simulink model "VFlexP"  (R2024a)
settings: Solver=ode23tb  StartTime=0.0  StopTime=3  FixedStep=1e-5
model workspace (MAT data in the model file):
  DCop_DCBUCK.op = opcond.OperatingPoint
  DCop_DCBUCK.op.Model_ = 'untitled4'
  DCop_DCBUCK.op.States_(1) = opcond.StatePoint
  DCop_DCBUCK.op.States_(1).Nx_ = 1
  DCop_DCBUCK.op.States_(1).Block_ = 'untitled4/DCBUCK/Integrator'
  DCop_DCBUCK.op.States_(1).x_ = 0.0993111458289
  DCop_DCBUCK.op.States_(2) = opcond.StatePoint
  DCop_DCBUCK.op.States_(2).Nx_ = 1
  DCop_DCBUCK.op.States_(2).Block_ = 'untitled4/DCBUCK/Integrator1'
  DCop_DCBUCK.op.States_(2).x_ = -1.0059432275
  DCop_DCBUCK.op_report = opcond.OperatingReport
  DCop_DCBUCK.op_report.Outputs_ = opcond.OutputReport
  DCop_DCBUCK.op_report.Outputs_.yspec_ = 0.0993111426985
  DCop_DCBUCK.op_report.Outputs_.Block_ = 'untitled4/out_trim1'
  DCop_DCBUCK.op_report.Outputs_.PortWidth_ = 1
  DCop_DCBUCK.op_report.Outputs_.PortNumber_ = NaN
  DCop_DCBUCK.op_report.Outputs_.y_ = 0.0993111458289
  DCop_DCBUCK.op_report.Outputs_.Known_ = 1
  DCop_DCBUCK.op_report.Outputs_.Min_ = -Inf
  DCop_DCBUCK.op_report.Outputs_.Max_ = Inf
  DCop_DCBUCK.op_report.TerminationString_ = 'Operating point specifications were successfully met.'
  DCop_DCBUCK.op_report.OptimizationOutput_.iterations = 1
  DCop_DCBUCK.op_report.OptimizationOutput_.funcCount = 6
  DCop_DCBUCK.op_report.OptimizationOutput_.constrviolation = 8.64996069397e-05
  DCop_DCBUCK.op_report.OptimizationOutput_.stepsize = 2.19887440386
  DCop_DCBUCK.op_report.OptimizationOutput_.algorithm = 'interior-point'
  DCop_DCBUCK.op_report.OptimizationOutput_.firstorderopt = 0
  DCop_DCBUCK.op_report.OptimizationOutput_.cgiterations = 0
  DCop_DCBUCK.op_report.OptimizationOutput_.message = 'Local minimum found that satisfies the constraints.
    | 
    | Optimization completed because the objective function is non-decreasing in 
    | feasible directions, to within the value of the optimality tolerance,
    | and constraints are satisfied to within the value of the constraint tolerance.
    | 
    | <stopping criteria details>
    | 
    | Optimization completed: The relative first-order optimality measure, 0.000000e+00,
    | is less than options.OptimalityTolerance = 1.000000e-06, and the relative maximum constraint
    | violation, 9.451558e-09, is less than options.ConstraintTolerance = 1.000000e-06.'
  DCop_DCBUCK.op_report.OptimizationOutput_.bestfeasible = []
  DCop_DCBUCK.op_report.Model_ = 'untitled4'
  DCop_DCBUCK.op_report.States_(1) = opcond.StateReport
  DCop_DCBUCK.op_report.States_(1).dx_ = 8.64996069397e-05
  DCop_DCBUCK.op_report.States_(1).Nx_ = 1
  DCop_DCBUCK.op_report.States_(1).Block_ = 'untitled4/DCBUCK/Integrator'
  DCop_DCBUCK.op_report.States_(1).x_ = 0.0993111458289
  DCop_DCBUCK.op_report.States_(1).SteadyState_ = 1
  DCop_DCBUCK.op_report.States_(1).dxMin_ = -Inf
  DCop_DCBUCK.op_report.States_(1).dxMax_ = Inf
  DCop_DCBUCK.op_report.States_(1).Known_ = 0
  DCop_DCBUCK.op_report.States_(1).Min_ = -Inf
  DCop_DCBUCK.op_report.States_(1).Max_ = Inf
  DCop_DCBUCK.op_report.States_(2) = opcond.StateReport
  DCop_DCBUCK.op_report.States_(2).dx_ = -1.77018447944e-06
  DCop_DCBUCK.op_report.States_(2).Nx_ = 1
  DCop_DCBUCK.op_report.States_(2).Block_ = 'untitled4/DCBUCK/Integrator1'
  DCop_DCBUCK.op_report.States_(2).x_ = -1.0059432275
  DCop_DCBUCK.op_report.States_(2).SteadyState_ = 1
  DCop_DCBUCK.op_report.States_(2).dxMin_ = -Inf
  DCop_DCBUCK.op_report.States_(2).dxMax_ = Inf
  DCop_DCBUCK.op_report.States_(2).Known_ = 0
  DCop_DCBUCK.op_report.States_(2).Min_ = -Inf
  DCop_DCBUCK.op_report.States_(2).Max_ = Inf
  Grid_CCVSC_idx = [2; 3; 4; 5; 6; 7; 8; 9; 10; 11; 12]
  Grid_CCVSCs = 1
  Grid_CCVSCs_buses = 1
  Grid_CCVSCs_toM = [0 1 0 0 0 0 0 0 0 0 0 0 ... (781 elements, 71x11)]
  Grid_C_Lines = [0 0]
  Grid_Cbuses = [0.00666666666667 0.00666666666667 0.00666666666667]
  Grid_DC.include = 1
  Grid_DC.Nbuses = 1
  Grid_DC.from = []
  Grid_DC.to = []
  Grid_DC.bus = 4
  Grid_DC.v = 1
  Grid_DC.Lines_toM = []
  Grid_DC.Lines_fromM = []
  Grid_DC.R_Lines = []
  Grid_DC.i_branch = []
  Grid_DC.Rbus = 150
  Grid_DC.DC_PESs_buses = 1
  Grid_DC.DC_PESs_toM = 1
  Grid_DC.DC_PESs_Pg = 0.0025
  Grid_DC.DC_VSMs_toM = [0; 0; 1]
  Grid_DC.DC_VSMs_DC_toM = 1
  Grid_DC.DC_VSMs_buses = 3
  Grid_DC.DC_VSMs_DC_buses = 1
  Grid_DC.DC_VSM_dparams.ratio = 1
  Grid_DC.DC_VSM_dparams.type = 1
  Grid_DC.DC_VSM_dparams.Rf = 0.0003
  Grid_DC.DC_VSM_dparams.Lf = 0.0355
  Grid_DC.DC_VSM_dparams.alpha1 = 0.001
  Grid_DC.DC_VSM_dparams.alpha2 = 0.0015
  Grid_DC.DC_VSM_dparams.alpha3 = 0.002
  Grid_DC.DC_VSM_dparams.Gsw = 0
  Grid_DCop_DCBUCK.op = opcond.OperatingPoint
  Grid_DCop_DCBUCK.op.Model_ = 'untitled'
  Grid_DCop_DCBUCK.op.States_(1) = opcond.StatePoint
  Grid_DCop_DCBUCK.op.States_(1).Nx_ = 1
  Grid_DCop_DCBUCK.op.States_(1).Block_ = 'untitled/DCBUCK/Integrator'
  Grid_DCop_DCBUCK.op.States_(1).x_ = 0.297042066445
  Grid_DCop_DCBUCK.op.States_(2) = opcond.StatePoint
  Grid_DCop_DCBUCK.op.States_(2).Nx_ = 1
  Grid_DCop_DCBUCK.op.States_(2).Block_ = 'untitled/DCBUCK/Integrator1'
  Grid_DCop_DCBUCK.op.States_(2).x_ = -1.00698752155
  Grid_DCop_DCBUCK.op_report = opcond.OperatingReport
  Grid_DCop_DCBUCK.op_report.Outputs_ = opcond.OutputReport
  Grid_DCop_DCBUCK.op_report.Outputs_.yspec_ = 0.297042068743
  Grid_DCop_DCBUCK.op_report.Outputs_.Block_ = 'untitled/out_trim1'
  Grid_DCop_DCBUCK.op_report.Outputs_.PortWidth_ = 1
  Grid_DCop_DCBUCK.op_report.Outputs_.PortNumber_ = NaN
  Grid_DCop_DCBUCK.op_report.Outputs_.y_ = 0.297042066445
  Grid_DCop_DCBUCK.op_report.Outputs_.Known_ = 1
  Grid_DCop_DCBUCK.op_report.Outputs_.Min_ = -Inf
  Grid_DCop_DCBUCK.op_report.Outputs_.Max_ = Inf
  Grid_DCop_DCBUCK.op_report.TerminationString_ = 'Operating point specifications were successfully met.'
  Grid_DCop_DCBUCK.op_report.OptimizationOutput_.iterations = 1
  Grid_DCop_DCBUCK.op_report.OptimizationOutput_.funcCount = 6
  Grid_DCop_DCBUCK.op_report.OptimizationOutput_.constrviolation = 8.27288844959e-05
  Grid_DCop_DCBUCK.op_report.OptimizationOutput_.stepsize = 2.12653445023
  Grid_DCop_DCBUCK.op_report.OptimizationOutput_.algorithm = 'interior-point'
  Grid_DCop_DCBUCK.op_report.OptimizationOutput_.firstorderopt = 0
  Grid_DCop_DCBUCK.op_report.OptimizationOutput_.cgiterations = 0
  Grid_DCop_DCBUCK.op_report.OptimizationOutput_.message = 'Local minimum found that satisfies the constraints.
    | 
    | Optimization completed because the objective function is non-decreasing in 
    | feasible directions, to within the value of the optimality tolerance,
    | and constraints are satisfied to within the value of the constraint tolerance.
    | 
    | <stopping criteria details>
    | 
    | Optimization completed: The relative first-order optimality measure, 0.000000e+00,
    | is less than options.OptimalityTolerance = 1.000000e-06, and the relative maximum constraint
    | violation, 8.342696e-09, is less than options.ConstraintTolerance = 1.000000e-06.'
  Grid_DCop_DCBUCK.op_report.OptimizationOutput_.bestfeasible = []
  Grid_DCop_DCBUCK.op_report.Model_ = 'untitled'
  Grid_DCop_DCBUCK.op_report.States_(1) = opcond.StateReport
  Grid_DCop_DCBUCK.op_report.States_(1).dx_ = 8.27288844959e-05
  Grid_DCop_DCBUCK.op_report.States_(1).Nx_ = 1
  Grid_DCop_DCBUCK.op_report.States_(1).Block_ = 'untitled/DCBUCK/Integrator'
  Grid_DCop_DCBUCK.op_report.States_(1).x_ = 0.297042066445
  Grid_DCop_DCBUCK.op_report.States_(1).SteadyState_ = 1
  Grid_DCop_DCBUCK.op_report.States_(1).dxMin_ = -Inf
  Grid_DCop_DCBUCK.op_report.States_(1).dxMax_ = Inf
  Grid_DCop_DCBUCK.op_report.States_(1).Known_ = 0
  Grid_DCop_DCBUCK.op_report.States_(1).Min_ = -Inf
  Grid_DCop_DCBUCK.op_report.States_(1).Max_ = Inf
  Grid_DCop_DCBUCK.op_report.States_(2) = opcond.StateReport
  Grid_DCop_DCBUCK.op_report.States_(2).dx_ = 1.29998784019e-06
  Grid_DCop_DCBUCK.op_report.States_(2).Nx_ = 1
  Grid_DCop_DCBUCK.op_report.States_(2).Block_ = 'untitled/DCBUCK/Integrator1'
  Grid_DCop_DCBUCK.op_report.States_(2).x_ = -1.00698752155
  Grid_DCop_DCBUCK.op_report.States_(2).SteadyState_ = 1
  Grid_DCop_DCBUCK.op_report.States_(2).dxMin_ = -Inf
  Grid_DCop_DCBUCK.op_report.States_(2).dxMax_ = Inf
  Grid_DCop_DCBUCK.op_report.States_(2).Known_ = 0
  Grid_DCop_DCBUCK.op_report.States_(2).Min_ = -Inf
  Grid_DCop_DCBUCK.op_report.States_(2).Max_ = Inf
  Grid_DCop_DC_PES.op = opcond.OperatingPoint
  Grid_DCop_DC_PES.op.Model_ = 'untitled1'
  Grid_DCop_DC_PES.op.States_(1) = opcond.StatePoint
  Grid_DCop_DC_PES.op.States_(1).Nx_ = 1
  Grid_DCop_DC_PES.op.States_(1).Block_ = 'untitled1/DC_PES/Integrator'
  Grid_DCop_DC_PES.op.States_(1).x_ = 0.166666683417
  Grid_DCop_DC_PES.op.States_(2) = opcond.StatePoint
  Grid_DCop_DC_PES.op.States_(2).Nx_ = 1
  Grid_DCop_DC_PES.op.States_(2).Block_ = 'untitled1/DC_PES/Integrator1'
  Grid_DCop_DC_PES.op.States_(2).x_ = 0.166666683333
  Grid_DCop_DC_PES.op_report = opcond.OperatingReport
  Grid_DCop_DC_PES.op_report.Outputs_ = opcond.OutputReport
  Grid_DCop_DC_PES.op_report.Outputs_.yspec_ = 0.166666666667
  Grid_DCop_DC_PES.op_report.Outputs_.Block_ = 'untitled1/out_trim1'
  Grid_DCop_DC_PES.op_report.Outputs_.PortWidth_ = 1
  Grid_DCop_DC_PES.op_report.Outputs_.PortNumber_ = NaN
  Grid_DCop_DC_PES.op_report.Outputs_.y_ = 0.166666683333
  Grid_DCop_DC_PES.op_report.Outputs_.Known_ = 1
  Grid_DCop_DC_PES.op_report.Outputs_.Min_ = -Inf
  Grid_DCop_DC_PES.op_report.Outputs_.Max_ = Inf
  Grid_DCop_DC_PES.op_report.TerminationString_ = 'Operating point specifications were successfully met.'
  Grid_DCop_DC_PES.op_report.OptimizationOutput_.iterations = 1
  Grid_DCop_DC_PES.op_report.OptimizationOutput_.funcCount = 6
  Grid_DCop_DC_PES.op_report.OptimizationOutput_.constrviolation = 1.66666662138e-08
  Grid_DCop_DC_PES.op_report.OptimizationOutput_.stepsize = 1.17851127835
  Grid_DCop_DC_PES.op_report.OptimizationOutput_.algorithm = 'interior-point'
  Grid_DCop_DC_PES.op_report.OptimizationOutput_.firstorderopt = 0
  Grid_DCop_DC_PES.op_report.OptimizationOutput_.cgiterations = 0
  Grid_DCop_DC_PES.op_report.OptimizationOutput_.message = 'Local minimum found that satisfies the constraints.
    | 
    | Optimization completed because the objective function is non-decreasing in 
    | feasible directions, to within the value of the optimality tolerance,
    | and constraints are satisfied to within the value of the constraint tolerance.
    | 
    | <stopping criteria details>
    | 
    | Optimization completed: The relative first-order optimality measure, 0.000000e+00,
    | is less than options.OptimalityTolerance = 1.000000e-06, and the relative maximum constraint
    | violation, 1.666667e-08, is less than options.ConstraintTolerance = 1.000000e-06.'
  Grid_DCop_DC_PES.op_report.OptimizationOutput_.bestfeasible.x = [0.166666683333; 0.166666683417]
  Grid_DCop_DC_PES.op_report.OptimizationOutput_.bestfeasible.fval = 0
  Grid_DCop_DC_PES.op_report.OptimizationOutput_.bestfeasible.constrviolation = 1.66666662138e-08
  Grid_DCop_DC_PES.op_report.OptimizationOutput_.bestfeasible.firstorderopt = 0
  Grid_DCop_DC_PES.op_report.Model_ = 'untitled1'
  Grid_DCop_DC_PES.op_report.States_(1) = opcond.StateReport
  Grid_DCop_DC_PES.op_report.States_(1).Nx_ = 1
  Grid_DCop_DC_PES.op_report.States_(1).Block_ = 'untitled1/DC_PES/Integrator'
  Grid_DCop_DC_PES.op_report.States_(1).x_ = 0.166666683417
  Grid_DCop_DC_PES.op_report.States_(1).SteadyState_ = 1
  Grid_DCop_DC_PES.op_report.States_(1).dxMin_ = -Inf
  Grid_DCop_DC_PES.op_report.States_(1).dxMax_ = Inf
  Grid_DCop_DC_PES.op_report.States_(1).Known_ = 0
  Grid_DCop_DC_PES.op_report.States_(1).Min_ = -Inf
  Grid_DCop_DC_PES.op_report.States_(1).Max_ = Inf
  Grid_DCop_DC_PES.op_report.States_(2) = opcond.StateReport
  Grid_DCop_DC_PES.op_report.States_(2).dx_ = 8.33333402284e-10
  Grid_DCop_DC_PES.op_report.States_(2).Nx_ = 1
  Grid_DCop_DC_PES.op_report.States_(2).Block_ = 'untitled1/DC_PES/Integrator1'
  Grid_DCop_DC_PES.op_report.States_(2).x_ = 0.166666683333
  Grid_DCop_DC_PES.op_report.States_(2).SteadyState_ = 1
  Grid_DCop_DC_PES.op_report.States_(2).dxMin_ = -Inf
  Grid_DCop_DC_PES.op_report.States_(2).dxMax_ = Inf
  Grid_DCop_DC_PES.op_report.States_(2).Known_ = 0
  Grid_DCop_DC_PES.op_report.States_(2).Min_ = -Inf
  Grid_DCop_DC_PES.op_report.States_(2).Max_ = Inf
  Grid_DFIGs = 1
  Grid_DFIGs_buses = 1
  Grid_DGs = "GFr"
  Grid_From_buses = [1 2]
  Grid_GFls = 1
  Grid_GFls_buses = 1
  Grid_GFr_idx = 1
  Grid_GFrs = 1
  Grid_GFrs_buses = 1
  Grid_GFrs_toM = [1; 0; 0]
  Grid_IG_idx = 2
  Grid_IGs = 1
  Grid_IGs_buses = 1
  Grid_IGs_toM = [0; 1]
  Grid_L_Lines = [0.05 0.05]
  Grid_L_Loads = 0
  Grid_Lines_fromM : object (value not decoded)
  Grid_Lines_toM : object (value not decoded)
  Grid_Load_buses = []
  Grid_Load_busesDC = []
  Grid_MSGs = 1
  Grid_MSGs_buses = 1
  Grid_Nbuses = 3
  Grid_PQ_gen = 3
  Grid_Ploads = []
  Grid_PloadsDC = []
  Grid_Ps_lf = -0.138475313333
  Grid_Qloads = []
  Grid_Qs_lf = 0.00594619333333
  Grid_R_Lines = [0.005 0.005]
  Grid_R_Loads = 0
  Grid_R_Loads_DC = 0
  Grid_Rcf = [150 150 150]
  Grid_SCs = 1
  Grid_SCs_buses = 1
  Grid_SG_idx = 1
  Grid_SGs = 1
  Grid_SGs_buses = 1
  Grid_SGs_toM = [1; 0]
  Grid_To_buses = [2 3]
  Grid_VCVSC_idx = [1; 2; 3; 4; 5; 6; 7; 8; 9; 10; 11; 12]
  Grid_VCVSCs = 1
  Grid_VCVSCs_buses = [1; 2; 3; 6; 8; 9; 12; 58; 59; 60; 63; 65]
  Grid_VCVSCs_toM = [1 0 0 0 0 0 0 0 0 0 0 0 ... (852 elements, 71x12)]
  Grid_VSM_idx = 2
  Grid_VSMs = 1
  Grid_VSMs_buses = 1
  Grid_VSMs_toM = [0; 1]
  Grid_admitt_matrix = [1.9801990198-19.801979198i  -1.9801980198+19.801980198i; -1.9801980198+19.801980198i  1.9801990198-19.801979198i]
  Grid_admitt_matrix_noloads = [1.9801990198-19.801979198i  -1.9801980198+19.801980198i; -1.9801980198+19.801980198i  1.9801990198-19.801979198i]
  Grid_bus = [1; 2; 3]
  Grid_busDC_complexity = 1
  Grid_busDC_complexity_PF = 2
  Grid_bus_complexity = [1 1 1]
  Grid_bus_complexity_PF = [1 1 1]
  Grid_buses_lf = 1
  Grid_conductance_matrix = 0.00666666666667
  Grid_conductance_matrix_noloads = 0.00666666666667
  Grid_fref.areas = 1
  Grid_fref.ref_units = 1
  Grid_fref.Fb_units = 1
  Grid_fref.buses = [1 1 1]
  Grid_fref.lines = [1 1]
  Grid_fref.loads = []
  Grid_fref.GFr = 1
  Grid_fref.DC_VSM = 1
  Grid_gen_static_params.mBase = 100
  Grid_iPs_lf = -7.22150378958
  Grid_iQs_lf = 168.17482109
  Grid_iadmitt_matrix = [250000.001075-249999.987531i  249999.998575-250000.012531i; 249999.998575-250000.012531i  250000.001075-249999.987531i]
  Grid_iadmitt_matrix_noloads = [250000.001075-249999.987531i  249999.998575-250000.012531i; 249999.998575-250000.012531i  250000.001075-249999.987531i]
  Grid_iconductance_matrix = 150
  Grid_iconductance_matrix_noloads = 150
  Grid_init_OK_bool = 1
  Grid_intconv_PF.include = 1
  Grid_intconv_PF.vmod = 1
  Grid_intconv_PF.vangle = 0.859745829367
  Grid_intconv_PF.P = -0.158700091527
  Grid_intconv_PF.Q = 0.0237163123873
  Grid_intconv_PF.from = [1 2 4]
  Grid_intconv_PF.to = [2 3 3]
  Grid_lf_op.op_report.Outputs(1).y = -0.138475313333
  Grid_lf_op.op_report.Outputs(2).y = 0.00594619333333
  Grid_lf_op.op_report.Outputs(3).y = [-0.145141982765 -0.151760481969]
  Grid_lf_op.op_report.Outputs(4).y = [-0.0126128600915 -0.0193289630611]
  Grid_lf_op.op_report.Outputs(5).y = [1 1.00009506691 0.999887421166]
  Grid_lf_op.op_report.Outputs(6).y = [0 0.00732016343869 0.0150048323525]
  Grid_lineDC_complexity = []
  Grid_lineDC_complexity_PF = []
  Grid_line_complexity = [1 1]
  Grid_line_complexity_PF = [3 3]
  Grid_loadDC_complexity = []
  Grid_loadDC_complexity_PF = []
  Grid_load_complexity = []
  Grid_load_complexity_PF = []
  Grid_opDC_CCVSC.P = [-0.000250314011939 0.0893885558248 -0.0965482172065 -0.839732591503 -0.318845576293 0.332848927017 0.493081958469 0.184553200933]
  Grid_opDC_CCVSC.Q = [-0.0188263035971 0.0721906871944 0.00896391516299 0.324071624692 -0.392719357789 -0.481473754372 -0.41568236758 -0.296587741983]
  Grid_opDC_CCVSC.id_out = [-0.000238257445549 0.0859724063763 -0.0913415354387 -0.807435184137 -0.305115384013 0.332898648568 0.502342982161 0.183243588375]
  Grid_opDC_CCVSC.iq_out = [0.0179195202435 -0.0694317861922 -0.00848050640623 -0.311607331434 0.375807997884 0.481545677758 0.423489678695 0.294483118332]
  Grid_opDC_CCVSC.PId = [-1.21511297231e-05 0.00657688908779 -0.00698762746106 -0.041179194391 -0.023341326877 0.0254667466155 0.0384292381353 0.0140181345107]
  Grid_opDC_CCVSC.PIq = [0.00091389553242 -0.00531153164371 -0.000648758740077 -0.0158919739032 0.0287493118381 0.0368382443485 0.0323969604201 0.0225279585524]
  Grid_opDC_CCVSC.frame = [-0.213709310357 -0.211881545906 -0.207881074849 0 -0.0555827722547 -0.0954948489365 -0.0996472270949 -0.073605567843]
  Grid_opDC_VSM.P = 0.158700091527
  Grid_opDC_VSM.Q = -0.0237163123873
  Grid_opDC_VSM.id_out = 0.158326365965
  Grid_opDC_VSM.iq_out = 0.0260949107001
  Grid_opDC_VSM.frame = 0.0206507879117
  Grid_opDC_VSM.id_in = 0.000111842024523
  Grid_opDC_VSM.iq_in = 1.84334910023e-05
  Grid_opDC_VSM.IP = 0
  Grid_opDC_VSM.iv = -0.000778396280495
  Grid_opGFr.Pd = -0.138475313333
  Grid_opGFr.Qd = 0.00594619333333
  Grid_opGFr.id_out = -0.138475313333
  Grid_opGFr.iq_out = -0.00594619333333
  Grid_opGFr.frame = -0.00139080832243
  Grid_opGFr.vd_c = 0.999921953718
  Grid_opGFr.vq_c = 0
  Grid_opGFr.iV = -7.80462817455e-05
  Grid_opGFr.v = 0.999921953718
  Grid_opGFr.IntConnect = 5
  Grid_opGFr.id_l = -0.138465909469
  Grid_opGFr.iq_l = 0.0938534152333
  Grid_opGFr.PIid = -0.00138465909469
  Grid_opGFr.PIiq = 0.000938534152333
  Grid_opGFr.PIvd = 9.99921953709e-06
  Grid_opGFr.PIvq = 0
  Grid_opVCVSC.Pd = 0
  Grid_opVCVSC.Qd = 0
  Grid_opVCVSC.id_out = [4.77012824674 0.000252372172029 0.387206076232 -0.00669815177796 4.43044477222 -0.00888398142826 2.79473009232 2.18798980312 0.322264460806 -0.0632019138679 -0.0604985051331 -0.0462539180443]
  Grid_opVCVSC.iq_out = [-1.25997186372 0.0149684790164 -0.231751502643 -0.0494644982143 -0.911066731256 -0.0589472249505 -1.80353640382 0.162268294537 -1.0981777606 -0.338765693762 -0.298705341855 -0.251695536875]
  Grid_opVCVSC.frame = [0.0438933282651 -0.0168438196467 -0.0841666076082 -0.134645533542 -0.017373173296 -0.149645793269 -0.137562101317 0.0572176344752 -0.0529798109092 -0.184784853699 -0.200116593784 -0.181975782571]
  Grid_opVCVSC.vd_c = [1.0583892424 1.00985029405 0.987381572831 0.980499160746 1.0168380704 0.980596131031 1.0316409122 1.06159711208 1.05617213999 1.01344616766 1.07304774652 1.09255913271]
  Grid_opVCVSC.vq_c = [6.93889390391e-18 3.46944695195e-18 0 2.77555756156e-17 0 -2.77555756156e-17 0 -6.93889390391e-18 6.93889390391e-18 -2.77555756156e-17 0 2.77555756156e-17]
  Grid_opVCVSC.iV = [0.0183892424009 -0.000149705952964 0.00238157283064 0.00049916074618 0.0118380704031 0.000596131030837 0.0166409121976 0.00159711208293 0.0111721399885 0.00344616765999 0.00304774652066 0.00255913270857]
  Grid_opVCVSC.v = [1.0583892424 1.00985029405 0.987381572831 0.980499160746 1.0168380704 0.980596131031 1.0316409122 1.06159711208 1.05617213999 1.01344616766 1.07304774652 1.09255913271]
  Grid_opVCVSC.id_l = [4.71024831855 1.231783245e-06 0.405319101793 3.52165566611e-06 4.44560451561 4.60461660484e-06 3.01564651745 2.19368980083 0.379967383234 0.000118194487427 8.76348532929e-05 6.10344572474e-05]
  Grid_opVCVSC.iq_l = [-1.36222896789 0.115955635796 -0.0996416062474 0.0481339685791 -0.732278422455 0.0384466913306 -1.30009716484 0.143039154495 -0.973954167095 -0.243266270257 -0.197465537031 -0.146654353471]
  Grid_opVCVSC.PIid = [0.000135655151574 3.5475357456e-11 1.16731901316e-05 1.01423683184e-10 0.00012803341005 1.32612958219e-10 8.68506197027e-05 6.31782662639e-05 1.09430606371e-05 3.40400123789e-09 2.52388377483e-09 1.75779236873e-09]
  Grid_opVCVSC.PIiq = [-3.92321942752e-05 3.33952231093e-06 -2.86967825993e-06 1.38625829508e-06 -2.10896185667e-05 1.10726471032e-06 -3.74427983473e-05 4.11952764945e-06 -2.80498800123e-05 -7.00606858342e-06 -5.68700746649e-06 -4.22364537998e-06]
  Grid_opVCVSC.PIvd = [3.67496264593e-05 3.50642463211e-05 3.42840823902e-05 3.40451097481e-05 3.53068774525e-05 3.40484767719e-05 3.58208650088e-05 3.68610108331e-05 3.66726437489e-05 3.51891030437e-05 3.72586023097e-05 3.79360809968e-05]
  Grid_opVCVSC.PIvq = [-3.85494105773e-15 0 0 0 4.81867632216e-16 0 -2.40933816108e-15 4.81867632216e-16 0 0 -4.81867632216e-16 -4.81867632216e-16]
  Grid_op_CCVSC.op = opcond.OperatingPoint
  Grid_op_CCVSC.op.Model_ = 'untitled'
  Grid_op_CCVSC.op.States_(1) = opcond.StatePoint
  Grid_op_CCVSC.op.States_(1).Nx_ = 11
  Grid_op_CCVSC.op.States_(1).Block_ = 'untitled/CCVSC/LPF/I'
  Grid_op_CCVSC.op.States_(1).x_ = [1.009861943; 0.981291076401; 0.971352962827; 1.00322239915; 0.969168759309; 1.00101830201; 1.05929040967; 1.04339572399; 0.992934596599; 1.04879026715; 1.07220457445]
  Grid_op_CCVSC.op.States_(2) = opcond.StatePoint
  Grid_op_CCVSC.op.States_(2).Nx_ = 11
  Grid_op_CCVSC.op.States_(2).Block_ = 'untitled/CCVSC/LPF1/I'
  Grid_op_CCVSC.op.States_(2).x_ = [-0.0166989844806; -0.085398033397; -0.129897735513; -0.0597487458922; -0.14529940151; -0.167892796173; 0.038779556309; -0.0578823653869; -0.184880740706; -0.211988173785; -0.196156450928]
  Grid_op_CCVSC.op.States_(3) = opcond.StatePoint
  Grid_op_CCVSC.op.States_(3).Nx_ = 11
  Grid_op_CCVSC.op.States_(3).Block_ = 'untitled/CCVSC/LPF2/I'
  Grid_op_CCVSC.op.States_(3).x_ = [1.009861943; 0.981291076401; 0.971352962827; 1.00322239915; 0.969168759309; 1.00101830201; 1.05929040967; 1.04339572399; 0.992934596599; 1.04879026715; 1.07220457445]
  Grid_op_CCVSC.op.States_(4) = opcond.StatePoint
  Grid_op_CCVSC.op.States_(4).Nx_ = 11
  Grid_op_CCVSC.op.States_(4).Block_ = 'untitled/CCVSC/LPF3/I'
  Grid_op_CCVSC.op.States_(4).x_ = [-0.0166989844806; -0.085398033397; -0.129897735513; -0.0597487458926; -0.14529940151; -0.167892796174; 0.0387795563087; -0.0578823653869; -0.184880740706; -0.211988173785; -0.196156450928]
  Grid_op_CCVSC.op.States_(5) = opcond.StatePoint
  Grid_op_CCVSC.op.States_(5).Nx_ = 11
  Grid_op_CCVSC.op.States_(5).Block_ = 'untitled/CCVSC/P'
  Grid_op_CCVSC.op.States_(5).x_ = [1.01727038409e-18; 0.400000000001; -1.80456749167e-13; 4.5000000022; 3.15175961175e-13; 3.10000001288; 2.32400000036; 0.400000000095; -1.95503794004e-12; -3.47571023681e-11; 9.07830100881e-12]
  Grid_op_CCVSC.op.States_(6) = opcond.StatePoint
  Grid_op_CCVSC.op.States_(6).Nx_ = 11
  Grid_op_CCVSC.op.States_(6).Block_ = 'untitled/CCVSC/PLL/dynamic/PLL/I'
  Grid_op_CCVSC.op.States_(6).x_ = [1; 1; 1; 0.999999999991; 1; 0.999999999962; 1; 1; 1; 1; 1]
  Grid_op_CCVSC.op.States_(7) = opcond.StatePoint
  Grid_op_CCVSC.op.States_(7).Nx_ = 11
  Grid_op_CCVSC.op.States_(7).Block_ = 'untitled/CCVSC/PLL/dynamic/frame'
  Grid_op_CCVSC.op.States_(7).x_ = [-0.0165344013704; -0.0868074935304; -0.132939939029; -0.0594865631615; -0.148813342999; -0.166175316605; 0.0365926525094; -0.0554181853462; -0.184088222665; -0.199439311658; -0.180945834503]
  Grid_op_CCVSC.op.States_(8) = opcond.StatePoint
  Grid_op_CCVSC.op.States_(8).Nx_ = 11
  Grid_op_CCVSC.op.States_(8).Block_ = 'untitled/CCVSC/Q'
  Grid_op_CCVSC.op.States_(8).x_ = [-0.015862822257; 0.120252486258; 0.0522438711347; 0.647307088531; 0.0546742450618; 1.36800880468; -0.0931237077542; 1.06159295924; 0.342624354062; 0.31755952052; 0.276277445204]
  Grid_op_CCVSC.op_report = opcond.OperatingReport
  Grid_op_CCVSC.op_report.Outputs_(1) = opcond.OutputReport
  Grid_op_CCVSC.op_report.Outputs_(1).yspec_ = [0.000259673583656; 0.393977793367; -0.0070661813362; 4.43140001829; -0.00827169417353; 2.7891744299; 2.18777108046; 0.325918162006; -0.0620965046483; -0.05879890244; -0.0456136713835]
  Grid_op_CCVSC.op_report.Outputs_(1).Block_ = 'untitled/out_trim1'
  Grid_op_CCVSC.op_report.Outputs_(1).PortWidth_ = 11
  Grid_op_CCVSC.op_report.Outputs_(1).PortNumber_ = NaN
  Grid_op_CCVSC.op_report.Outputs_(1).y_ = [0.000259673583656; 0.393977793229; -0.00706618133531; 4.43139980848; -0.00827169417363; 2.78917339713; 2.18777105686; 0.325918157997; -0.0620965045362; -0.0587989014357; -0.0456136713993]
  Grid_op_CCVSC.op_report.Outputs_(1).Known_ = [1; 1; 1; 1; 1; 1; 1; 1; 1; 1; 1]
  Grid_op_CCVSC.op_report.Outputs_(1).Min_ = [-Inf; -Inf; -Inf; -Inf; -Inf; -Inf; -Inf; -Inf; -Inf; -Inf; -Inf]
  Grid_op_CCVSC.op_report.Outputs_(1).Max_ = [Inf; Inf; Inf; Inf; Inf; Inf; Inf; Inf; Inf; Inf; Inf]
  Grid_op_CCVSC.op_report.Outputs_(2) = opcond.OutputReport
  Grid_op_CCVSC.op_report.Outputs_(2).yspec_ = [0.0157036177884; -0.156831564843; -0.0528396907676; -0.909148054024; -0.0551734384103; -1.8344231967; 0.16800352209; -1.03552070385; -0.3335002201; -0.290901679261; -0.24932744737]
  Grid_op_CCVSC.op_report.Outputs_(2).Block_ = 'untitled/out_trim2'
  Grid_op_CCVSC.op_report.Outputs_(2).PortWidth_ = 11
  Grid_op_CCVSC.op_report.Outputs_(2).PortNumber_ = NaN
  Grid_op_CCVSC.op_report.Outputs_(2).y_ = [0.0157036177884; -0.156831564765; -0.0528396907661; -0.909148031788; -0.0551734384082; -1.83442292878; 0.168003502174; -1.03552070255; -0.333500219896; -0.29090167819; -0.249327447093]
  Grid_op_CCVSC.op_report.Outputs_(2).Known_ = [1; 1; 1; 1; 1; 1; 1; 1; 1; 1; 1]
  Grid_op_CCVSC.op_report.Outputs_(2).Min_ = [-Inf; -Inf; -Inf; -Inf; -Inf; -Inf; -Inf; -Inf; -Inf; -Inf; -Inf]
  Grid_op_CCVSC.op_report.Outputs_(2).Max_ = [Inf; Inf; Inf; Inf; Inf; Inf; Inf; Inf; Inf; Inf; Inf]
  Grid_op_CCVSC.op_report.TerminationString_ = 'Operating point specifications were successfully met.'
  Grid_op_CCVSC.op_report.OptimizationOutput_.iterations = 3
  Grid_op_CCVSC.op_report.OptimizationOutput_.funcCount = 356
  Grid_op_CCVSC.op_report.OptimizationOutput_.constrviolation = 2.89733602665e-05
  Grid_op_CCVSC.op_report.OptimizationOutput_.stepsize = 8.75730946062e-07
  Grid_op_CCVSC.op_report.OptimizationOutput_.algorithm = 'interior-point'
  Grid_op_CCVSC.op_report.OptimizationOutput_.firstorderopt = 0
  Grid_op_CCVSC.op_report.OptimizationOutput_.cgiterations = 0
  Grid_op_CCVSC.op_report.OptimizationOutput_.message = 'Local minimum found that satisfies the constraints.
    | 
    | Optimization completed because the objective function is non-decreasing in 
    | feasible directions, to within the value of the optimality tolerance,
    | and constraints are satisfied to within the value of the constraint tolerance.
    | 
    | <stopping criteria details>
    | 
    | Optimization completed: The relative first-order optimality measure, 0.000000e+00,
    | is less than options.OptimalityTolerance = 1.000000e-06, and the relative maximum constraint
    | violation, 6.438525e-07, is less than options.ConstraintTolerance = 1.000000e-06.'
  Grid_op_CCVSC.op_report.OptimizationOutput_.bestfeasible = []
  Grid_op_CCVSC.op_report.Model_ = 'untitled'
  Grid_op_CCVSC.op_report.States_(1) = opcond.StateReport
  Grid_op_CCVSC.op_report.States_(1).dx_ = [0; -8.881784197e-14; 3.33066907388e-14; 2.35367281221e-12; 6.66133814775e-14; -9.1748830755e-11; 8.881784197e-13; -6.12843109593e-12; 2.33146835171e-13; 1.04360964315e-12; -2.22044604925e-14]
  Grid_op_CCVSC.op_report.States_(1).Nx_ = 11
  Grid_op_CCVSC.op_report.States_(1).Block_ = 'untitled/CCVSC/LPF/I'
  Grid_op_CCVSC.op_report.States_(1).x_ = [1.009861943; 0.981291076401; 0.971352962827; 1.00322239915; 0.969168759309; 1.00101830201; 1.05929040967; 1.04339572399; 0.992934596599; 1.04879026715; 1.07220457445]
  Grid_op_CCVSC.op_report.States_(1).SteadyState_ = [1; 1; 1; 1; 1; 1; 1; 1; 1; 1; 1]
  Grid_op_CCVSC.op_report.States_(1).dxMin_ = [-Inf; -Inf; -Inf; -Inf; -Inf; -Inf; -Inf; -Inf; -Inf; -Inf; -Inf]
  Grid_op_CCVSC.op_report.States_(1).dxMax_ = [Inf; Inf; Inf; Inf; Inf; Inf; Inf; Inf; Inf; Inf; Inf]
  Grid_op_CCVSC.op_report.States_(1).Known_ = [0; 0; 0; 0; 0; 0; 0; 0; 0; 0; 0]
  Grid_op_CCVSC.op_report.States_(1).Min_ = [-Inf; -Inf; -Inf; -Inf; -Inf; -Inf; -Inf; -Inf; -Inf; -Inf; -Inf]
  Grid_op_CCVSC.op_report.States_(1).Max_ = [Inf; Inf; Inf; Inf; Inf; Inf; Inf; Inf; Inf; Inf; Inf]
  Grid_op_CCVSC.op_report.States_(2) = opcond.StateReport
  Grid_op_CCVSC.op_report.States_(2).dx_ = [0; 3.85802501057e-13; 3.80251385934e-13; -3.1668417888e-11; 4.27435864481e-13; -1.02551300785e-10; -2.89226975703e-11; 5.26662047307e-13; -9.99200722163e-14; -2.40363284831e-12; -1.34614541736e-12]
  Grid_op_CCVSC.op_report.States_(2).Nx_ = 11
  Grid_op_CCVSC.op_report.States_(2).Block_ = 'untitled/CCVSC/LPF1/I'
  Grid_op_CCVSC.op_report.States_(2).x_ = [-0.0166989844806; -0.085398033397; -0.129897735513; -0.0597487458922; -0.14529940151; -0.167892796173; 0.038779556309; -0.0578823653869; -0.184880740706; -0.211988173785; -0.196156450928]
  Grid_op_CCVSC.op_report.States_(2).SteadyState_ = [1; 1; 1; 1; 1; 1; 1; 1; 1; 1; 1]
  Grid_op_CCVSC.op_report.States_(2).dxMin_ = [-Inf; -Inf; -Inf; -Inf; -Inf; -Inf; -Inf; -Inf; -Inf; -Inf; -Inf]
  Grid_op_CCVSC.op_report.States_(2).dxMax_ = [Inf; Inf; Inf; Inf; Inf; Inf; Inf; Inf; Inf; Inf; Inf]
  Grid_op_CCVSC.op_report.States_(2).Known_ = [0; 0; 0; 0; 0; 0; 0; 0; 0; 0; 0]
  Grid_op_CCVSC.op_report.States_(2).Min_ = [-Inf; -Inf; -Inf; -Inf; -Inf; -Inf; -Inf; -Inf; -Inf; -Inf; -Inf]
  Grid_op_CCVSC.op_report.States_(2).Max_ = [Inf; Inf; Inf; Inf; Inf; Inf; Inf; Inf; Inf; Inf; Inf]
  Grid_op_CCVSC.op_report.States_(3) = opcond.StateReport
  Grid_op_CCVSC.op_report.States_(3).dx_ = [0; -3.7627989613e-08; -4.49945636305e-09; -4.6817306476e-06; -4.84622342256e-09; -2.89733602665e-05; -1.25802135376e-06; -2.23016383138e-07; -7.25810522795e-08; -5.29354471368e-07; -1.1638969788e-07]
  Grid_op_CCVSC.op_report.States_(3).Nx_ = 11
  Grid_op_CCVSC.op_report.States_(3).Block_ = 'untitled/CCVSC/LPF2/I'
  Grid_op_CCVSC.op_report.States_(3).x_ = [1.009861943; 0.981291076401; 0.971352962827; 1.00322239915; 0.969168759309; 1.00101830201; 1.05929040967; 1.04339572399; 0.992934596599; 1.04879026715; 1.07220457445]
  Grid_op_CCVSC.op_report.States_(3).SteadyState_ = [1; 1; 1; 1; 1; 1; 1; 1; 1; 1; 1]
  Grid_op_CCVSC.op_report.States_(3).dxMin_ = [-Inf; -Inf; -Inf; -Inf; -Inf; -Inf; -Inf; -Inf; -Inf; -Inf; -Inf]
  Grid_op_CCVSC.op_report.States_(3).dxMax_ = [Inf; Inf; Inf; Inf; Inf; Inf; Inf; Inf; Inf; Inf; Inf]
  Grid_op_CCVSC.op_report.States_(3).Known_ = [0; 0; 0; 0; 0; 0; 0; 0; 0; 0; 0]
  Grid_op_CCVSC.op_report.States_(3).Min_ = [-Inf; -Inf; -Inf; -Inf; -Inf; -Inf; -Inf; -Inf; -Inf; -Inf; -Inf]
  Grid_op_CCVSC.op_report.States_(3).Max_ = [Inf; Inf; Inf; Inf; Inf; Inf; Inf; Inf; Inf; Inf; Inf]
  Grid_op_CCVSC.op_report.States_(4) = opcond.StateReport
  Grid_op_CCVSC.op_report.States_(4).dx_ = [0; -3.13662568141e-09; -1.01869901403e-09; 7.20071362953e-07; 2.0284746105e-09; 1.545790487e-05; 8.24665298549e-07; 3.50140891281e-07; -9.12854514201e-09; -1.88931087441e-07; 5.35036820404e-08]
  Grid_op_CCVSC.op_report.States_(4).Nx_ = 11
  Grid_op_CCVSC.op_report.States_(4).Block_ = 'untitled/CCVSC/LPF3/I'
  Grid_op_CCVSC.op_report.States_(4).x_ = [-0.0166989844806; -0.085398033397; -0.129897735513; -0.0597487458926; -0.14529940151; -0.167892796174; 0.0387795563087; -0.0578823653869; -0.184880740706; -0.211988173785; -0.196156450928]
  Grid_op_CCVSC.op_report.States_(4).SteadyState_ = [1; 1; 1; 1; 1; 1; 1; 1; 1; 1; 1]
  Grid_op_CCVSC.op_report.States_(4).dxMin_ = [-Inf; -Inf; -Inf; -Inf; -Inf; -Inf; -Inf; -Inf; -Inf; -Inf; -Inf]
  Grid_op_CCVSC.op_report.States_(4).dxMax_ = [Inf; Inf; Inf; Inf; Inf; Inf; Inf; Inf; Inf; Inf; Inf]
  Grid_op_CCVSC.op_report.States_(4).Known_ = [0; 0; 0; 0; 0; 0; 0; 0; 0; 0; 0]
  Grid_op_CCVSC.op_report.States_(4).Min_ = [-Inf; -Inf; -Inf; -Inf; -Inf; -Inf; -Inf; -Inf; -Inf; -Inf; -Inf]
  Grid_op_CCVSC.op_report.States_(4).Max_ = [Inf; Inf; Inf; Inf; Inf; Inf; Inf; Inf; Inf; Inf; Inf]
  Grid_op_CCVSC.op_report.States_(5) = opcond.StateReport
  Grid_op_CCVSC.op_report.States_(5).dx_ = [-8.42021724855e-19; -1.03750341651e-11; 1.8066117432e-12; -2.1979271736e-08; -3.14934577617e-12; -1.28780199837e-07; -3.59431151509e-09; -9.4528940231e-10; 1.95485394618e-11; 3.47507380102e-10; -9.08167885259e-11]
  Grid_op_CCVSC.op_report.States_(5).Nx_ = 11
  Grid_op_CCVSC.op_report.States_(5).Block_ = 'untitled/CCVSC/P'
  Grid_op_CCVSC.op_report.States_(5).x_ = [1.01727038409e-18; 0.400000000001; -1.80456749167e-13; 4.5000000022; 3.15175961175e-13; 3.10000001288; 2.32400000036; 0.400000000095; -1.95503794004e-12; -3.47571023681e-11; 9.07830100881e-12]
  Grid_op_CCVSC.op_report.States_(5).SteadyState_ = [1; 1; 1; 1; 1; 1; 1; 1; 1; 1; 1]
  Grid_op_CCVSC.op_report.States_(5).dxMin_ = [-Inf; -Inf; -Inf; -Inf; -Inf; -Inf; -Inf; -Inf; -Inf; -Inf; -Inf]
  Grid_op_CCVSC.op_report.States_(5).dxMax_ = [Inf; Inf; Inf; Inf; Inf; Inf; Inf; Inf; Inf; Inf; Inf]
  Grid_op_CCVSC.op_report.States_(5).Known_ = [0; 0; 0; 0; 0; 0; 0; 0; 0; 0; 0]
  Grid_op_CCVSC.op_report.States_(5).Min_ = [-Inf; -Inf; -Inf; -Inf; -Inf; -Inf; -Inf; -Inf; -Inf; -Inf; -Inf]
  Grid_op_CCVSC.op_report.States_(5).Max_ = [Inf; Inf; Inf; Inf; Inf; Inf; Inf; Inf; Inf; Inf; Inf]
  Grid_op_CCVSC.op_report.States_(6) = opcond.StateReport
  Grid_op_CCVSC.op_report.States_(6).dx_ = [0; 2.68729483111e-12; 3.79418718666e-12; 8.72443783884e-11; 4.44810854816e-12; 3.83996723308e-10; 1.44183276429e-12; 5.59829960167e-13; 7.40518757425e-13; -1.09456887998e-11; -1.15710219184e-11]
  Grid_op_CCVSC.op_report.States_(6).Nx_ = 11
  Grid_op_CCVSC.op_report.States_(6).Block_ = 'untitled/CCVSC/PLL/dynamic/PLL/I'
  Grid_op_CCVSC.op_report.States_(6).x_ = [1; 1; 1; 0.999999999991; 1; 0.999999999962; 1; 1; 1; 1; 1]
  Grid_op_CCVSC.op_report.States_(6).SteadyState_ = [1; 1; 1; 1; 1; 1; 1; 1; 1; 1; 1]
  Grid_op_CCVSC.op_report.States_(6).dxMin_ = [-Inf; -Inf; -Inf; -Inf; -Inf; -Inf; -Inf; -Inf; -Inf; -Inf; -Inf]
  Grid_op_CCVSC.op_report.States_(6).dxMax_ = [Inf; Inf; Inf; Inf; Inf; Inf; Inf; Inf; Inf; Inf; Inf]
  Grid_op_CCVSC.op_report.States_(6).Known_ = [0; 0; 0; 0; 0; 0; 0; 0; 0; 0; 0]
  Grid_op_CCVSC.op_report.States_(6).Min_ = [-Inf; -Inf; -Inf; -Inf; -Inf; -Inf; -Inf; -Inf; -Inf; -Inf; -Inf]
  Grid_op_CCVSC.op_report.States_(6).Max_ = [Inf; Inf; Inf; Inf; Inf; Inf; Inf; Inf; Inf; Inf; Inf]
  Grid_op_CCVSC.op_report.States_(7) = opcond.StateReport
  Grid_op_CCVSC.op_report.States_(7).dx_ = [0; 0; 0; 0; 6.97573699602e-14; 9.13821546478e-12; 6.97573699602e-14; 6.97573699602e-14; 0; 1.11611791936e-12; -4.18544219761e-13]
  Grid_op_CCVSC.op_report.States_(7).Nx_ = 11
  Grid_op_CCVSC.op_report.States_(7).Block_ = 'untitled/CCVSC/PLL/dynamic/frame'
  Grid_op_CCVSC.op_report.States_(7).x_ = [-0.0165344013704; -0.0868074935304; -0.132939939029; -0.0594865631615; -0.148813342999; -0.166175316605; 0.0365926525094; -0.0554181853462; -0.184088222665; -0.199439311658; -0.180945834503]
  Grid_op_CCVSC.op_report.States_(7).SteadyState_ = [1; 1; 1; 1; 1; 1; 1; 1; 1; 1; 1]
  Grid_op_CCVSC.op_report.States_(7).dxMin_ = [-Inf; -Inf; -Inf; -Inf; -Inf; -Inf; -Inf; -Inf; -Inf; -Inf; -Inf]
  Grid_op_CCVSC.op_report.States_(7).dxMax_ = [Inf; Inf; Inf; Inf; Inf; Inf; Inf; Inf; Inf; Inf; Inf]
  Grid_op_CCVSC.op_report.States_(7).Known_ = [0; 0; 0; 0; 0; 0; 0; 0; 0; 0; 0]
  Grid_op_CCVSC.op_report.States_(7).Min_ = [-Inf; -Inf; -Inf; -Inf; -Inf; -Inf; -Inf; -Inf; -Inf; -Inf; -Inf]
  Grid_op_CCVSC.op_report.States_(7).Max_ = [Inf; Inf; Inf; Inf; Inf; Inf; Inf; Inf; Inf; Inf; Inf]
  Grid_op_CCVSC.op_report.States_(8) = opcond.StateReport
  Grid_op_CCVSC.op_report.States_(8).dx_ = [-3.46944695195e-17; -6.46714626296e-11; -7.22963355848e-12; -8.82571127292e-09; -7.94676824345e-12; -5.54142687292e-08; -2.61821259118e-10; -4.6777914875e-10; -1.31483157695e-10; -9.21122622621e-10; -2.07436290367e-10]
  Grid_op_CCVSC.op_report.States_(8).Nx_ = 11
  Grid_op_CCVSC.op_report.States_(8).Block_ = 'untitled/CCVSC/Q'
  Grid_op_CCVSC.op_report.States_(8).x_ = [-0.015862822257; 0.120252486258; 0.0522438711347; 0.647307088531; 0.0546742450618; 1.36800880468; -0.0931237077542; 1.06159295924; 0.342624354062; 0.31755952052; 0.276277445204]
  Grid_op_CCVSC.op_report.States_(8).SteadyState_ = [1; 1; 1; 1; 1; 1; 1; 1; 1; 1; 1]
  Grid_op_CCVSC.op_report.States_(8).dxMin_ = [-Inf; -Inf; -Inf; -Inf; -Inf; -Inf; -Inf; -Inf; -Inf; -Inf; -Inf]
  Grid_op_CCVSC.op_report.States_(8).dxMax_ = [Inf; Inf; Inf; Inf; Inf; Inf; Inf; Inf; Inf; Inf; Inf]
  Grid_op_CCVSC.op_report.States_(8).Known_ = [0; 0; 0; 0; 0; 0; 0; 0; 0; 0; 0]
  Grid_op_CCVSC.op_report.States_(8).Min_ = [-Inf; -Inf; -Inf; -Inf; -Inf; -Inf; -Inf; -Inf; -Inf; -Inf; -Inf]
  Grid_op_CCVSC.op_report.States_(8).Max_ = [Inf; Inf; Inf; Inf; Inf; Inf; Inf; Inf; Inf; Inf; Inf]
  Grid_op_IG.op = opcond.OperatingPoint
  Grid_op_IG.op.Model_ = 'untitled1'
  Grid_op_IG.op.States_(1) = opcond.StatePoint
  Grid_op_IG.op.States_(1).Nx_ = 1
  Grid_op_IG.op.States_(1).Block_ = 'untitled1/IG/Integrator1'
  Grid_op_IG.op.States_(1).x_ = 0.820913653733
  Grid_op_IG.op.States_(2) = opcond.StatePoint
  Grid_op_IG.op.States_(2).Nx_ = 1
  Grid_op_IG.op.States_(2).Block_ = 'untitled1/IG/Integrator2'
  Grid_op_IG.op.States_(2).x_ = -0.571050962271
  Grid_op_IG.op.States_(3) = opcond.StatePoint
  Grid_op_IG.op.States_(3).Nx_ = 1
  Grid_op_IG.op.States_(3).Block_ = 'untitled1/IG/PQ/LPF_P/I'
  Grid_op_IG.op.States_(3).x_ = -0.895923909342
  Grid_op_IG.op.States_(4) = opcond.StatePoint
  Grid_op_IG.op.States_(4).Nx_ = 1
  Grid_op_IG.op.States_(4).Block_ = 'untitled1/IG/PQ/LPF_Q/I'
  Grid_op_IG.op.States_(4).x_ = 0.110165648811
  Grid_op_IG.op.States_(5) = opcond.StatePoint
  Grid_op_IG.op.States_(5).Nx_ = 1
  Grid_op_IG.op.States_(5).Block_ = 'untitled1/IG/RL out/dynamic/i_d'
  Grid_op_IG.op.States_(5).x_ = -0.88566290577
  Grid_op_IG.op.States_(6) = opcond.StatePoint
  Grid_op_IG.op.States_(6).Nx_ = 1
  Grid_op_IG.op.States_(6).Block_ = 'untitled1/IG/RL out/dynamic/i_q'
  Grid_op_IG.op.States_(6).x_ = -0.174405673219
  Grid_op_IG.op.States_(7) = opcond.StatePoint
  Grid_op_IG.op.States_(7).Nx_ = 1
  Grid_op_IG.op.States_(7).Block_ = 'untitled1/IG/theta'
  Grid_op_IG.op.States_(7).x_ = 0.67986934424
  Grid_op_IG.op_report = opcond.OperatingReport
  Grid_op_IG.op_report.Outputs_(1) = opcond.OutputReport
  Grid_op_IG.op_report.Outputs_(1).yspec_ = -0.885662905776
  Grid_op_IG.op_report.Outputs_(1).Block_ = 'untitled1/out_trim1'
  Grid_op_IG.op_report.Outputs_(1).PortWidth_ = 1
  Grid_op_IG.op_report.Outputs_(1).PortNumber_ = NaN
  Grid_op_IG.op_report.Outputs_(1).y_ = -0.88566290577
  Grid_op_IG.op_report.Outputs_(1).Known_ = 1
  Grid_op_IG.op_report.Outputs_(1).Min_ = -Inf
  Grid_op_IG.op_report.Outputs_(1).Max_ = Inf
  Grid_op_IG.op_report.Outputs_(2) = opcond.OutputReport
  Grid_op_IG.op_report.Outputs_(2).yspec_ = -0.17440567322
  Grid_op_IG.op_report.Outputs_(2).Block_ = 'untitled1/out_trim2'
  Grid_op_IG.op_report.Outputs_(2).PortWidth_ = 1
  Grid_op_IG.op_report.Outputs_(2).PortNumber_ = NaN
  Grid_op_IG.op_report.Outputs_(2).y_ = -0.174405673219
  Grid_op_IG.op_report.Outputs_(2).Known_ = 1
  Grid_op_IG.op_report.Outputs_(2).Min_ = -Inf
  Grid_op_IG.op_report.Outputs_(2).Max_ = Inf
  Grid_op_IG.op_report.TerminationString_ = 'Operating point specifications were successfully met.'
  Grid_op_IG.op_report.OptimizationOutput_.iterations = 5
  Grid_op_IG.op_report.OptimizationOutput_.funcCount = 48
  Grid_op_IG.op_report.OptimizationOutput_.constrviolation = 0.0135829750943
  Grid_op_IG.op_report.OptimizationOutput_.stepsize = 9.02072851792e-06
  Grid_op_IG.op_report.OptimizationOutput_.algorithm = 'interior-point'
  Grid_op_IG.op_report.OptimizationOutput_.firstorderopt = 0
  Grid_op_IG.op_report.OptimizationOutput_.cgiterations = 0
  Grid_op_IG.op_report.OptimizationOutput_.message = 'Local minimum found that satisfies the constraints.
    | 
    | Optimization completed because the objective function is non-decreasing in 
    | feasible directions, to within the value of the optimality tolerance,
    | and constraints are satisfied to within the value of the constraint tolerance.
    | 
    | <stopping criteria details>
    | 
    | Optimization completed: The relative first-order optimality measure, 0.000000e+00,
    | is less than options.OptimalityTolerance = 1.000000e-06, and the relative maximum constraint
    | violation, 3.301086e-11, is less than options.ConstraintTolerance = 1.000000e-06.'
  Grid_op_IG.op_report.OptimizationOutput_.bestfeasible = []
  Grid_op_IG.op_report.Model_ = 'untitled1'
  Grid_op_IG.op_report.States_(1) = opcond.StateReport
  Grid_op_IG.op_report.States_(1).Nx_ = 1
  Grid_op_IG.op_report.States_(1).Block_ = 'untitled1/IG/Integrator1'
  Grid_op_IG.op_report.States_(1).x_ = 0.820913653733
  Grid_op_IG.op_report.States_(1).SteadyState_ = 1
  Grid_op_IG.op_report.States_(1).dxMin_ = -Inf
  Grid_op_IG.op_report.States_(1).dxMax_ = Inf
  Grid_op_IG.op_report.States_(1).Known_ = 0
  Grid_op_IG.op_report.States_(1).Min_ = -Inf
  Grid_op_IG.op_report.States_(1).Max_ = Inf
  Grid_op_IG.op_report.States_(2) = opcond.StateReport
  Grid_op_IG.op_report.States_(2).Nx_ = 1
  Grid_op_IG.op_report.States_(2).Block_ = 'untitled1/IG/Integrator2'
  Grid_op_IG.op_report.States_(2).x_ = -0.571050962271
  Grid_op_IG.op_report.States_(2).SteadyState_ = 1
  Grid_op_IG.op_report.States_(2).dxMin_ = -Inf
  Grid_op_IG.op_report.States_(2).dxMax_ = Inf
  Grid_op_IG.op_report.States_(2).Known_ = 0
  Grid_op_IG.op_report.States_(2).Min_ = -Inf
  Grid_op_IG.op_report.States_(2).Max_ = Inf
  Grid_op_IG.op_report.States_(3) = opcond.StateReport
  Grid_op_IG.op_report.States_(3).dx_ = -2.22044604925e-14
  Grid_op_IG.op_report.States_(3).Nx_ = 1
  Grid_op_IG.op_report.States_(3).Block_ = 'untitled1/IG/PQ/LPF_P/I'
  Grid_op_IG.op_report.States_(3).x_ = -0.895923909342
  Grid_op_IG.op_report.States_(3).SteadyState_ = 1
  Grid_op_IG.op_report.States_(3).dxMin_ = -Inf
  Grid_op_IG.op_report.States_(3).dxMax_ = Inf
  Grid_op_IG.op_report.States_(3).Known_ = 0
  Grid_op_IG.op_report.States_(3).Min_ = -Inf
  Grid_op_IG.op_report.States_(3).Max_ = Inf
  Grid_op_IG.op_report.States_(4) = opcond.StateReport
  Grid_op_IG.op_report.States_(4).dx_ = -1.66533453694e-14
  Grid_op_IG.op_report.States_(4).Nx_ = 1
  Grid_op_IG.op_report.States_(4).Block_ = 'untitled1/IG/PQ/LPF_Q/I'
  Grid_op_IG.op_report.States_(4).x_ = 0.110165648811
  Grid_op_IG.op_report.States_(4).SteadyState_ = 1
  Grid_op_IG.op_report.States_(4).dxMin_ = -Inf
  Grid_op_IG.op_report.States_(4).dxMax_ = Inf
  Grid_op_IG.op_report.States_(4).Known_ = 0
  Grid_op_IG.op_report.States_(4).Min_ = -Inf
  Grid_op_IG.op_report.States_(4).Max_ = Inf
  Grid_op_IG.op_report.States_(5) = opcond.StateReport
  Grid_op_IG.op_report.States_(5).dx_ = -0.0135829750943
  Grid_op_IG.op_report.States_(5).Nx_ = 1
  Grid_op_IG.op_report.States_(5).Block_ = 'untitled1/IG/RL out/dynamic/i_d'
  Grid_op_IG.op_report.States_(5).x_ = -0.88566290577
  Grid_op_IG.op_report.States_(5).SteadyState_ = 1
  Grid_op_IG.op_report.States_(5).dxMin_ = -Inf
  Grid_op_IG.op_report.States_(5).dxMax_ = Inf
  Grid_op_IG.op_report.States_(5).Known_ = 0
  Grid_op_IG.op_report.States_(5).Min_ = -Inf
  Grid_op_IG.op_report.States_(5).Max_ = Inf
  Grid_op_IG.op_report.States_(6) = opcond.StateReport
  Grid_op_IG.op_report.States_(6).dx_ = -0.00752599858976
  Grid_op_IG.op_report.States_(6).Nx_ = 1
  Grid_op_IG.op_report.States_(6).Block_ = 'untitled1/IG/RL out/dynamic/i_q'
  Grid_op_IG.op_report.States_(6).x_ = -0.174405673219
  Grid_op_IG.op_report.States_(6).SteadyState_ = 1
  Grid_op_IG.op_report.States_(6).dxMin_ = -Inf
  Grid_op_IG.op_report.States_(6).dxMax_ = Inf
  Grid_op_IG.op_report.States_(6).Known_ = 0
  Grid_op_IG.op_report.States_(6).Min_ = -Inf
  Grid_op_IG.op_report.States_(6).Max_ = Inf
  Grid_op_IG.op_report.States_(7) = opcond.StateReport
  Grid_op_IG.op_report.States_(7).Nx_ = 1
  Grid_op_IG.op_report.States_(7).Block_ = 'untitled1/IG/theta'
  Grid_op_IG.op_report.States_(7).x_ = 0.67986934424
  Grid_op_IG.op_report.States_(7).SteadyState_ = 1
  Grid_op_IG.op_report.States_(7).dxMin_ = -Inf
  Grid_op_IG.op_report.States_(7).dxMax_ = Inf
  Grid_op_IG.op_report.States_(7).Known_ = 0
  Grid_op_IG.op_report.States_(7).Min_ = -Inf
  Grid_op_IG.op_report.States_(7).Max_ = Inf
  Grid_op_SG : object (value not decoded)
  Grid_op_VSM : object (value not decoded)
  Grid_shift_lines = [0 0]
  Grid_tap_lines = [1 1]
  Grid_v_buses_mod = [1 1.0001218564 1]
  LinsysParamChangeStruct : Param1 (value not decoded)
  Lline = 0.01
  Rline = 1e-05
  linsys : object (value not decoded)
symbols that are objects in the model workspace (value not decoded): Grid_op_SG, Grid_op_VSM
undefined symbols (not defined in the file or in its folder): block_buses_DC, block_idx, CCVSC_idx, Cf, costs, costs2, DFIGs_nodes, DiscIntNeverNeededParam, entity, Fb, Fi, From_nodes, Grid_op_DFIG, Grid_op_DFIG_PQ, Grid_op_MSG, Grid_op_SC, Grid_op_VCVSC, Kic, Kiv, Kpc, Kpv, last_send, Lc, Lf, m, Matrix_flux_to_i, mD, mp, MSGs_buses, Nbuses_DC, nq, op_VCVSC, Psche, Rc, Rf, rkq1, rkq2, SCs_buses, SCs_nodes, sec_control_structure, set_DG_up, set_extra_satur, set_sending_cost, SGs_buses, SGs_nodes, Tf, To_nodes, VI_L, VI_R, WOF_Tf, xkq1, xkq2
libraries: simulink x447, eeGeneralControl x5
(part 1 of 30)
settings Model: Creator=atomas  LastModifiedBy=atomas
settings SolverCC: ZeroCrossControl=DisableAll
settings DataIOCC: InitialState=getstatestruct(op1)  SaveFormat=StructureWithTime
settings OptimizationCC: ReuseModelBlockBuffer=off
settings DebuggingCC: ReadBeforeWriteMsg=DisableAll  WriteAfterWriteMsg=DisableAll  WriteAfterReadMsg=DisableAll  AlgebraicLoopMsg=none  MultiTaskDSMMsg=none  UnderSpecifiedDimensionMsg=warning
settings ModelReferenceCC: UpdateModelReferenceTargets=IfOutOfDate
settings SFSimCC: SFSimEcho=off
settings RTWCC: GPUComputeCapability=3.5

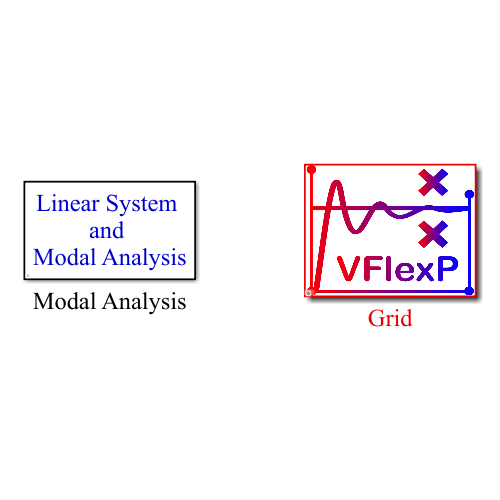
[thumbnail: Simulink's stored preview of the top-level diagram]
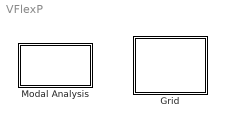
== system VFlexP ==
  Grid : Subsystem  Variant=on  VariantControlMode=label  VariantControl=Choice  LabelModeActiveChoice=Dynamic  mask(Grid){bvarname=Grid_, Sb=0.015, Fb_data={'1','50'}, bus_data={'1','3','0','0','0.0001','0.0001','1','1.0000000000','0.0000000000','230','1','1.1','0.9','dynamic','series RL static omega','dynamic','PQ';'2','1','0','0','0.0001','0.0001','1','1.0001218564','0.4193671127','230','1','1.1','0.9','dynamic','series RL static omega','dynamic','PQ';'3','1','0','0','0.0001','0.0001','1','1.0000000000','0.8597458294','230','1','1.1','0.9','dynamic','series RL static omega','dynamic','PQ';'4','1','0','0','0.0001','0','2','1.0000000000','1.1832029910','230','1','1.1','0.9','DC dynamic','DC ConstR','dynamic','PQ'}, gen_data={'1','GFr','-0.0020771297','0.0000891929','1000','-1000','1','100','1','1000','-100','0','0','0','0','0','0','0','0','0','0','0';'4','DC_PES','0.0025000000','0.0000000000','1000','-1000','1','100','1','1000','-100','0','0','0','0','0','0','0','0','0','0','0'}, line_data={'1','2','0.005','0.05','0','0','0','0','0','0','1','-360','360','dynamic','static omega';'2','3','0.005','0.05','0','0','0','0','0','0','1','-360','360','dynamic','static omega'}, save_in_workspace=off, parameter_change_filename=1, param_change_data={}, SC_structure=No SC, define_SC_in_MATLAB=on, delayM=0, passM=1, A_f_sc=1, A_P_sc=1, A_v_sc=1, A_Q_sc=1, g_f_sc=1, g_P_sc=1, g_v_sc=1, g_Q_sc=1, intconv_data={'DC_VSM','4','3','0.0003','0.0355','0','1000','1000','1000','1','0','1','-360','360','0','0','0','0','0','0','0','0','1','1','1.22','0.75','1','0','1','-0.5','0.5','-360','360','0','0.001','0.0015','0.002','0'}, TC_structure=No TC}
      mask prompts: Sb "Base power (MW)"; Fb_data "Base frequency (Hz)"; save_in_workspace "Save in Workspace"; parameter_change_filename "Filename "Parameter_Change_V_""; SC_structure "Secondary control structure"; define_SC_in_MATLAB "Define control structure in MATLAB"; TC_structure "Tertiary control structure"
      mask init:
      | bvarname = [matlab.lang.makeValidName(get_param(gcb, 'Name')) '_'];
      |     set_param(gcb, "bvarname", bvarname)
      |     mdlWks = get_param(bdroot,'ModelWorkspace'); % Get the model workspace
      | 
      |     % Initialise variables
      |     v_buses_mod = [];
      |     Cbuses = [];
      |     DGs = [];
      |     From_buses = [];
      |     L_Lines = [];
      |     shift_lines = [];
      |     tap_lines = [];
      |     L_Loads = [];
      |     Load_buses = [];
      |     Nbuses = [];
      |     PQ_gen = [];
      |     Ploads = [];
      |     Ps_lf = [];
      |     Qloads = [];
      |     Qs_lf = [];
      |     R_Lines = [];
      |     C_Lines = [];
      |     R_Loads = [];
      |     Rcf = [];
      |     To_buses = [];
      |     Lines_fromM = [];
      |     Lines_toM = [];
      |     iPs_lf = [];
      |     iQs_lf = [];
      |     bus = [];
      |     buses_lf = [];
      |     line_complexity = [];
      |     bus_complexity = [];
      |     load_complexity = [];
      |     line_complexity_PF = [];
      |     bus_complexity_PF = [];
      |     load_complexity_PF = [];
      |     admitt_matrix = [];
      |     iadmitt_matrix = [];
      |     admitt_matrix_noloads = [];
      |     iadmitt_matrix_noloads = [];
      |     gen_static_params = [];
      |     gen_to_plot = 1;
      |     loadDC_complexity = [];
      |     lineDC_complexity = [];
      |     busDC_complexity = [];
      |     loadDC_complexity_PF = [];
      |     lineDC_complexity_PF = [];
      |     busDC_complexity_PF = [];
      |     fref.ref_units = 1;
      |     omega_base = 2*pi*50;
      | 
      |     bl = find_system([gcb '/Dynamic/Generators'], ...
      |         'IncludeCommented', 'on', 'SearchDepth', '2', ...
      |         'LookUnderMasks', 'on', 'Name', 'trim_output');
      |     for i = 1:length(bl) 
      |        DG_namei = get_param(get_param(bl{i}, 'Parent'), 'Name');
      |        eval([DG_namei 's = [];']);
      |        eval([DG_namei 's_buses = 1;']);
      |        eval([DG_namei '_idx = [];']);
      |     end
      | 
      |     try
      |         v_buses_mod = mdlWks.getVariable([bvarname 'v_buses_mod']);
      |         Cbuses = mdlWks.getVariable([bvarname 'Cbuses']);
      |         DGs = mdlWks.getVariable([bvarname 'DGs']);
      |         gen_static_params = mdlWks.getVariable([bvarname 'gen_static_params']);
      |         From_buses = mdlWks.getVariable([bvarname 'From_buses']);
      |         L_Lines = mdlWks.getVariable([bvarname 'L_Lines']);
      |         tap_lines = mdlWks.getVariable([bvarname 'tap_lines']);
      |         shift_lines = mdlWks.getVariable([bvarname 'shift_lines']);
      |         L_Loads = mdlWks.getVariable([bvarname 'L_Loads']);
      |         Load_buses = mdlWks.getVariable([bvarname 'Load_buses']);
      |         Load_busesDC = mdlWks.getVariable([bvarname 'Load_busesDC']);
      |         Nbuses = mdlWks.getVariable([bvarname 'Nbuses']);
      |         PQ_gen = mdlWks.getVariable([bvarname 'PQ_gen']);
      |         Ploads = mdlWks.getVariable([bvarname 'Ploads']);
      |         Ps_lf = mdlWks.getVariable([bvarname 'Ps_lf']);
      |         Qloads = mdlWks.getVariable([bvarname 'Qloads']);
      |         Qs_lf = mdlWks.getVariable([bvarname 'Qs_lf']);
      |         R_Lines = mdlWks.getVariable([bvarname 'R_Lines']);
      |         C_Lines = mdlWks.getVariable([bvarname 'C_Lines']);
      |         R_Loads = mdlWks.getVariable([bvarname 'R_Loads']);
      |         Rcf = mdlWks.getVariable([bvarname 'Rcf']);
      |         To_buses = mdlWks.getVariable([bvarname 'To_buses']);
      |         Lines_fromM = mdlWks.getVariable([bvarname 'Lines_fromM']);
      |         Lines_toM = mdlWks.getVariable([bvarname 'Lines_toM']);
      |         iPs_lf = mdlWks.getVariable([bvarname 'iPs_lf']);
      |         iQs_lf = mdlWks.getVariable([bvarname 'iQs_lf']);
      |         bus = mdlWks.getVariable([bvarname 'bus']);
      |         buses_lf = mdlWks.getVariable([bvarname 'buses_lf']);
      |         PloadsDC = mdlWks.getVariable([bvarname 'PloadsDC']);
      |         R_Loads_DC = mdlWks.getVariable([bvarname 'R_Loads_DC']);
      |         line_complexity = mdlWks.getVariable([bvarname 'line_complexity']);
      |         bus_complexity = mdlWks.getVariable([bvarname 'bus_complexity']);
      |         load_complexity = mdlWks.getVariable([bvarname 'load_complexity']);
      |         line_complexity_PF = mdlWks.getVariable([bvarname 'line_complexity_PF']);
      |         bus_complexity_PF = mdlWks.getVariable([bvarname 'bus_complexity_PF']);
      |         load_complexity_PF = mdlWks.getVariable([bvarname 'load_complexity_PF']);
      |         loadDC_complexity = mdlWks.getVariable([bvarname 'loadDC_complexity']);
      |         loadDC_complexity_PF = mdlWks.getVariable([bvarname 'loadDC_complexity_PF']);
      |         lineDC_complexity = mdlWks.getVariable([bvarname 'lineDC_complexity']);
      |         lineDC_complexity_PF = mdlWks.getVariable([bvarname 'lineDC_complexity_PF']);
      |         busDC_complexity = mdlWks.getVariable([bvarname 'busDC_complexity']);
      |         busDC_complexity_PF = mdlWks.getVariable([bvarname 'busDC_complexity_PF']);
      |         admitt_matrix = mdlWks.getVariable([bvarname 'admitt_matrix']);
      |         iadmitt_matrix = mdlWks.getVariable([bvarname 'iadmitt_matrix']);
      |         admitt_matrix_noloads = mdlWks.getVariable([bvarname 'admitt_matrix_noloads']);
      |         iadmitt_matrix_noloads = mdlWks.getVariable([bvarname 'iadmitt_matrix_noloads']);
      |         conductance_matrix = mdlWks.getVariable([bvarname 'conductance_matrix']);
      |         iconductance_matrix = mdlWks.getVariable([bvarname 'iconductance_matrix']);
      |         conductance_matrix_noloads = mdlWks.getVariable([bvarname 'conductance_matrix_noloads']);
      |         iconductance_matrix_noloads = mdlWks.getVariable([bvarname 'iconductance_matrix_noloads']);
      |         
      |         if length(buses_lf) <= 25
      |             gen_to_plot = 1:length(buses_lf);
      |         end
      |         for i = 1:length(bl)
      |            try
      |                DG_namei = get_param(get_param(bl{i}, 'Parent'), 'Name');
      |                aux1 = mdlWks.getVariable([bvarname DG_namei 's']);
      |                aux2 = mdlWks.getVariable([bvarname DG_namei 's_buses']);
      |                aux4 = mdlWks.getVariable([bvarname DG_namei '_idx']);
      |                eval([DG_namei 's = aux1;']);
      |                eval([DG_namei 's_buses = aux2;']);
      |                eval([DG_namei '_idx = aux4;']);
      |            catch
      |            end
      |         end
      |     if strcmp(get_param(gcb, "LabelModeActiveChoice"), "Dynamic") ...
      |                 && (strcmp(get_param([gcb '/Dynamic/Secondary Control'], ...
      |                 "LabelModeActiveChoice"), "Matrices")...
      |                 || strcmp(get_param([gcb '/Dynamic/Secondary Control'], ...
      |                 "LabelModeActiveChoice"), "Matrices1")...
      |                 || strcmp(get_param([gcb '/Dynamic/Secondary Control'], ...
      |                 "LabelModeActiveChoice"), "Matrices with delay")) ...
      |                 && ~define_SC_in_MATLAB
      |         DGs_number = length(buses_lf);
      |         delayM = 0.1*circshift(eye(DGs_number), 1);
      |         passM = circshift(eye(DGs_number), 1);
      |         A_f_sc = circshift(eye(DGs_number), 1);
      |         A_P_sc = circshift(eye(DGs_number), 1);
      |         A_v_sc = eye(DGs_number);
      |         A_Q_sc = circshift(eye(DGs_number), 1);
      |         A_f_sc(1,:) = 0;
      |         A_P_sc(1,:) = 0;
      |         A_v_sc(1,:) = 0;
      |         A_Q_sc(1,:) = 0;
      |         A_f_sc(1,1) = 0; % Leader follows reference frequency
      |         A_P_sc(1,1) = 1; % Leader is slack
      |         A_Q_sc(1,1) = 1; % Leader is slack
      |         g_f_sc = zeros(1, DGs_number);
      |         g_P_sc = zeros(1, DGs_number);
      |         g_v_sc = zeros(1, DGs_number);
      |         g_Q_sc = zeros(1, DGs_number);
      |         g_f_sc(1) = 1; % Leader follows reference frequency
      |         g_v_sc(1) = 1; % Leader follows reference voltage
      |     elseif strcmp(get_param(gcb, "LabelModeActiveChoice"), "Dynamic") ...
      |                 && strcmp(get_param([gcb '/Dynamic/Secondary Control'], ...
      |                 "LabelModeActiveChoice"), ...
      |                 "Matrices with delay and limitation") && ~define_SC_in_MATLAB
      |         DGs_number = length(buses_lf);
      |         delayM = 0*0.1*circshift(eye(DGs_number), 1);
      |         passM = circshift(eye(DGs_number), 1);
      |         A_f_sc = circshift(eye(DGs_number), 1);
      |         A_P_sc = circshift(eye(DGs_number), 1);
      |         A_v_sc = circshift(eye(DGs_number), 1);
      |         A_Q_sc = circshift(eye(DGs_number), 1);
      |         g_f_sc = zeros(1, DGs_number);
      |         g_P_sc = zeros(1, DGs_number);
      |         g_v_sc = zeros(1, DGs_number);
      |         g_Q_sc = zeros(1, DGs_number);
      |         g_f_sc(1) = 1; % Leader follows reference frequency
      |         g_v_sc(1) = 1; % Leader follows reference voltage
      |     end
      | 
      |     catch ME
      |         %errordlg(ME.message)
      |     end
      |     try
      |         DC = mdlWks.getVariable([bvarname 'DC']);
      |         intconv_PF = mdlWks.getVariable([bvarname 'intconv_PF']);
      |         fref = mdlWks.getVariable([bvarname 'fref']);
      |         omega_base = 2*pi*cell2mat(Fb_data(:,2))';
      |     catch ME
      |         %errordlg(ME.message)
      |     end
      mask Help: web('doc_Home.html')
      mask Callback bus_data: fun_bus_data_callback(gcb)
      mask Callback gen_data: fun_gen_data_callback(gcb)
      mask Callback line_data: fun_line_data_callback(gcb)
      mask Callback param_change_data: fun_apply_changes_block(gcb)
      mask TypeOptions SC_structure: No SC | Pilot nodes | Matrices | Matrices1 | Matrices with delay | Matrices with delay and limitation | MAS UC | MAS UC binary | MAS messages
      mask Callback SC_structure:
      | set_param([gcb '/Dynamic/Secondary Control'],...
      |     'LabelModeActiveChoice', ...
      |     get_param(gcb, "SC_structure"))
      mask Callback define_SC_in_MATLAB:
      | p = Simulink.Mask.get(gcb); param = p.getDialogControl('tSC_table');
      | if strcmp(get_param(gcb, "define_SC_in_MATLAB"), 'off')
      |     param.Visible = 'off';
      | else
      |     param.Visible = 'on';
      | end
      mask Callback intconv_data: fun_intconv_data_callback(gcb)
      mask TypeOptions TC_structure: No TC | MAS edp | MAS messages | Scheduled
      mask Callback TC_structure:
      | set_param([gcb '/Dynamic/Tertiary Control'],...
      |     'LabelModeActiveChoice', ...
      |     get_param(gcb, "TC_structure"))
      mask DialogControl load_system Prompt: Load system
      mask DialogControl load_system Callback: fun_load_system_callback(gcb)
      mask DialogControl save_table Prompt: Save table file
      mask DialogControl save_table Callback: fun_save_table_callback(gcb)
      mask DialogControl MATPOWER_loadflow Prompt: MATPOWER Loadflow
      mask DialogControl MATPOWER_loadflow Callback: fun_MATPOWER_loadflow(gcb)
      mask DialogControl loadflow Prompt: Loadflow
      mask DialogControl loadflow Callback: fun_loadflow_callback(gcb)
      mask DialogControl lf_report Prompt: Loadflow report
      mask DialogControl lf_report Callback: fun_lf_report_callback(gcb)
      mask DialogControl init_units Prompt: Initialise units
      mask DialogControl init_units Callback: fun_init_units_callback(gcb)
      mask DialogControl load_complexity Prompt: Load complexity in grid
      mask DialogControl load_complexity Callback: fun_load_complexity_grid(gcb)
      mask DialogControl Scope_gen Prompt: Show generators signals
      mask DialogControl Scope_gen Callback: open_system([gcb '/Dynamic/Scope_gen'])
      mask DialogControl simulate_simulink Prompt: Simulate
      mask DialogControl simulate_simulink Callback:
      | model = bdroot;
      | sim(model);
      mask DialogControl Control34 Prompt: Instituto de Investigación Tecnológica. <br> Universidad Pontificia Comillas.
      mask DialogControl Control34 Callback: web('https://www.iit.comillas.edu/')
      mask DialogControl home_tab Prompt: System parameters
      mask DialogControl new_row_Fb Prompt: +
      mask DialogControl new_row_Fb Callback: fun_mask_new_row_Fb(gcb)
      mask DialogControl delete_row_Fb Prompt: -
      mask DialogControl delete_row_Fb Callback: fun_mask_delete_row_Fb(gcb)
      mask DialogControl clear_Fb_table Prompt: Clear
      mask DialogControl clear_Fb_table Callback:
      | maskObj = Simulink.Mask.get(gcb);
      |     tableControl = maskObj.getDialogControl( 'Fb_data' );
      |     for i=1:tableControl.getNumberOfRows()
      |         tableControl.removeRow(1);
      |     end
      mask DialogControl bus_tab Prompt: Bus data
      mask DialogControl new_row_bus Prompt: +
      mask DialogControl new_row_bus Callback: fun_mask_new_row_Bus(gcb)
      mask DialogControl delete_row_bus Prompt: -
      mask DialogControl delete_row_bus Callback: fun_mask_delete_row_Bus(gcb)
      mask DialogControl clear_bus_table Prompt: Clear
      mask DialogControl clear_bus_table Callback:
      | maskObj = Simulink.Mask.get(gcb);
      |     tableControl = maskObj.getDialogControl( 'bus_data' );
      |     for i=1:tableControl.getNumberOfRows()
      |         tableControl.removeRow(1);
      |     end
      mask DialogControl gen_tab Prompt: Gen data
      mask DialogControl refresh_DGs Prompt: Refresh DG options
      mask DialogControl refresh_DGs Callback: fun_refresh_DGs_callback(gcb)
      mask DialogControl open_DG Prompt: Open DGs configuration
      mask DialogControl open_DG Callback: fun_open_DG_callback(gcb)
      mask DialogControl new_row_gen Prompt: +
      mask DialogControl new_row_gen Callback: fun_mask_new_row_Gen(gcb)
      mask DialogControl delete_row_gen Prompt: -
      mask DialogControl delete_row_gen Callback: fun_mask_delete_row_Gen(gcb)
      mask DialogControl clear_gen_table Prompt: Clear
      mask DialogControl clear_gen_table Callback:
      | maskObj = Simulink.Mask.get(gcb);
      |     tableControl = maskObj.getDialogControl( 'gen_data' );
      |     for i=1:tableControl.getNumberOfRows()
      |         tableControl.removeRow(1);
      |     end
      mask DialogControl line_tab Prompt: Line data
      mask DialogControl new_row_line Prompt: +
      mask DialogControl new_row_line Callback: fun_mask_new_row_Line(gcb)
      mask DialogControl delete_row_line Prompt: -
      mask DialogControl delete_row_line Callback: fun_mask_delete_row_Line(gcb)
      mask DialogControl clear_line_table Prompt: Clear
      mask DialogControl clear_line_table Callback:
      | maskObj = Simulink.Mask.get(gcb);
      |     tableControl = maskObj.getDialogControl( 'line_data' );
      |     for i=1:tableControl.getNumberOfRows()
      |         tableControl.removeRow(1);
      |     end
      mask DialogControl param_change Prompt: Parameter Variation
      mask DialogControl execute_parameter_change Prompt: Execute Parameter Change
      mask DialogControl execute_parameter_change Callback: fun_execute_parameter_change(gcb)
      mask DialogControl new_parameter Prompt: +
      mask DialogControl new_parameter Callback: fun_mask_new_row_Param(gcb)
      mask DialogControl delete_parameter Prompt: -
      mask DialogControl delete_parameter Callback: fun_mask_delete_row_Param(gcb)
      mask DialogControl clear_param_table Prompt: Clear
      mask DialogControl clear_param_table Callback:
      | maskObj = Simulink.Mask.get(gcb);
      |     tableControl = maskObj.getDialogControl( 'param_change_data' );
      |     for i=1:tableControl.getNumberOfRows()
      |         tableControl.removeRow(1);
      |     end
      mask DialogControl plot_change_parameter Prompt: Plot Selected Parameter
      mask DialogControl plot_change_parameter Callback: fun_plot_change_parameter_callback(gcb)
      mask DialogControl Secondary_control Prompt: Secondary control
      mask DialogControl Construct_MAS Prompt: Construct_MAS
      mask DialogControl Construct_MAS Callback: fun_construct_MAS_callback(gcb)
      mask DialogControl Initialise_0 Prompt: Initialise all variables to 0
      mask DialogControl Initialise_0 Callback: fun_initialise_0_callback(gcb)
      mask DialogControl intconv_tab Prompt: Int converters
      mask DialogControl new_row_intconv Prompt: +
      mask DialogControl new_row_intconv Callback: fun_mask_new_row_Intconv(gcb)
      mask DialogControl delete_row_intconv Prompt: -
      mask DialogControl delete_row_intconv Callback: fun_mask_delete_row_Intconv(gcb)
      mask DialogControl clear_intconv_tabl Prompt: Clear
      mask DialogControl clear_intconv_tabl Callback:
      | maskObj = Simulink.Mask.get(gcb);
      |     tableControl = maskObj.getDialogControl( 'intconv_data' );
      |     for i=1:tableControl.getNumberOfRows()
      |         tableControl.removeRow(1);
      |     end
      mask DialogControl Tertiary_control Prompt: Tertiary control
      mask DialogControl Construct_MAS_tertiary Prompt: Construct_MAS
      mask DialogControl Construct_MAS_tertiary Callback: fun_construct_MAS_callback(gcb)
      mask DialogControl Initialise_0_copy Prompt: Initialise all variables to 0
      mask DialogControl Initialise_0_copy Callback: fun_initialise_0_callback(gcb)
      mask Display: image('$imagefile');
  Modal Analysis : Subsystem
      mask Help: web([extractBefore(get_param(bdroot, 'FileName'), ['\' gcs '.slx']) '\Documentation\modal_analysis.html'])
      mask DialogControl DescTextVar Prompt: FAST MODAL ANALYSIS TOOL
      mask DialogControl ParameterGroupVar Prompt: ANALYSIS
      mask DialogControl calculate_linsys Prompt: Calculate Linear System
      mask DialogControl calculate_linsys Callback:
      | wb = waitbar(0, 'Linearizing the system', 'Name','Linear System Option'); % Waitbar
      |     model = bdroot;
      |     io = getlinio(model);
      |     waitbar(0.25,wb)
      |     try
      |         linsys = linearize(model,io);
      |          waitbar(0.5,wb)
      |         if height(linsys)>1
      |             linsys = linsys(1,1);
      |         end
      |             waitbar(0.75,wb)
      |         modelworkspace=get_param(model,"ModelWorkspace");
      | 
      |         assignin("base","linsys",linsys);
      |         assignin(modelworkspace,"linsys",linsys);
      |         waitbar(1,wb)
      | 
      |     catch
      |         try
      |         waitbar(0.5,wb)
      |         linsys = linearize(model,io);
      |         waitbar(0.75,wb)
      |         if height(linsys)>1
      |             linsys = linsys(1,1);
      |         end
      |         waitbar(1,wb)
      |         modelworkspace=get_param(model,"ModelWorkspace");
      | 
      |         assignin("base","linsys",linsys);
      |         assignin(modelworkspace,"linsys",linsys);
      |         catch ME
      |              msg = ["There has being a problem calculating the modal analysis",...
      |             "Please check:"," - (1) you are working on the simulink model folder",...
      |             " - (2) The scripts for the linearized trigonometric functions are " + ...
      |             "in the same folder",...
      |             " - (3) There is still one input perturbation and one output measurement in the system"];
      |             errordlg(msg);
      |             errordlg(ME.message);
      |         end
      |     end
      | 
      |     close(wb)
      mask DialogControl modal_analysis_calculation Prompt: Modal Analysis Excel Generator
      mask DialogControl modal_analysis_calculation Callback:
      | wb = waitbar(0, 'Modal Analisys', 'Name','Exporting Modal Analysis Caculation'); % Waitbar
      | 
      |     model = bdroot;
      |     waitbar(0.25,wb)
      |     modelworkspace=get_param(model,"ModelWorkspace");
      |     linsys = evalin(modelworkspace,"linsys");
      |   if ~isempty(linsys)
      |         A = linsys.a;
      |       [v,z] = eig(A);
      |         n = height(A);
      |         % Eigenvalues
      |         z = diag(z) ;
      |         %[magz,iz]=sort(1./abs(z));
      |         [~,iz]=sort(1./imag(z));
      |         z = z(iz);
      |         v = v(:,iz);
      |         % Right eigenvectors
      |         for i = 1:n
      |           [~,imax] = max(abs(v(:,i))) ;
      |           v(:,i) = v(:,i)/v(imax,i) ;
      |         end
      |         % Left eigenvectors
      |         w=inv(v);
      |         % Participations
      |         for i = 1:n
      |           for j = 1:n
      |             p(i,j) = w(j,i)*v(i,j);
      |           end
      |         end
      |                 Xvec_vars = linsys.StateName;
      | 
      |     waitbar(0.5,wb)
      | 
      |     N = height(A);
      |     nombrevar = char(Xvec_vars);
      | 
      |     Variables_Names = char(nombrevar);
      |     Modes = string(1:N)';
      |     T1 = table(Variables_Names);
      |     T =  array2table(abs(p));
      |     T.Properties.VariableNames = Modes;
      |     TPart = [T1 T];
      |     waitbar(0.6,wb)
      | 
      |     TeigenvaluesTitle = ({'Eigenvalue'; 'REAL';'IMAGINARY';'DAMPING';'FREQUENCY'});
      |     Eig_Table = [ array2table([ (1:length(z))' real(z) imag(z) -real(z)./abs(z)*100,abs(z)./2/pi])];
      |     Eig_Table.Properties.VariableNames = TeigenvaluesTitle;
      |     waitbar(0.7,wb)
      | 
      |     unstable_eigenvalues = find(real(z)>0);
      | 
      |      if unstable_eigenvalues>1
      |         TPart_Unstable = sortrows([T1 TPart(:,unstable_eigenvalues+1)],2,{'descend'});
      |      end
      |     else
      |         msg = "There has being a problem calculating the modal analysis";
      |         f = warndlg(msg);
      |     end
      |     try
      |         filename ="ModalAnalysisTables.xlsx";
      |         writetable(sortrows(Eig_Table,4,{'ascend'}),filename,"Sheet","SUMMARY BY DAMPING");
      |         writetable(sortrows(Eig_Table,5,{'ascend'}),filename,"Sheet","SUMMARY BY FREQUENCY");
      |     waitbar(0.8,wb)
      | 
      |         writetable(TPart,filename,"Sheet","Participations");
      |         if (unstable_eigenvalues)>1
      |             writetable(TPart_Unstable,filename,"Sheet","Unstable Participations");
      |         else
      |             writematrix([0 0],filename,"Sheet","Unstable Participations");
      |         end
      |         writematrix([real(v) imag(v)],filename,"Sheet","Left Eigenvectors");
      |         waitbar(0.9,wb)
      | 
      |         writematrix([real(w) imag(w)],filename,"Sheet","Right Eigenvectors");
      |         waitbar(1,wb)
      | 
      |         msg = "TABLES HAVE BEEN CORRECTLY EXPORTED";
      |         f = warndlg(msg);
      |     catch
      |          msg = ["TABLES COULD NOT BE MADE"," MAKE SURE THE EXCEL IS CLOSED"];
      |          f = warndlg(msg);
      | 
      | 
      |     end
      |         close(wb)
      mask DialogControl plot_eigenvalues Prompt: Plot EigenValues
      mask DialogControl plot_eigenvalues Callback:
      | model = bdroot;
      | 
      |     modelworkspace=get_param(model,"ModelWorkspace");
      |     linsys = evalin(modelworkspace,"linsys");
      | 
      |     figure(1);clf;
      |     plot(real(eig(linsys.a)),imag(eig(linsys.a)),'*');
      |     grid on
      mask DialogControl plot_eigenvalues_mod_angle Prompt: Plot Eigenvalues Mod&Angle
      mask DialogControl plot_eigenvalues_mod_angle Callback:
      | model = bdroot;
      | 
      | modelworkspace=get_param(model,"ModelWorkspace");
      | linsys = evalin(modelworkspace,"linsys");
      | figure(1);clf;
      | loglog(abs(eig(linsys.a)),rad2deg(wrapTo2Pi(angle(eig(linsys.a)))),'*');
      | 
      | xlimit = log10(xlim); %ylimit = ylim;
      | 
      | for i=logspace(2*xlimit(1)-xlimit(2),xlimit(2),40)
      |     line(min(max(i./abs(cos(deg2rad(90:1:270))),0.99*10^xlimit(1)), ...
      |     1.01*10^xlimit(2)),90:1:270,'LineStyle','-','Color','black','HandleVisibility','off');
      | end
      | 
      | ylim([90-20 180])
      mask DialogControl run_andres_tool Prompt: Advanced Simulink Modal Analysis Tool
      mask DialogControl run_andres_tool Callback: simulink_modal_analysis(bdroot);
      mask DialogControl Container3 Prompt: CLEAR SYSTEMS
      mask DialogControl clear_simulink Prompt: Clear SIMULINK Workspace
      mask DialogControl clear_simulink Callback:
      | model = bdroot;
      |     command_clear = "clear all";
      | 
      |     modelworkspace=get_param(model,"ModelWorkspace");
      |     evalin(modelworkspace,command_clear)
      mask DialogControl clear_matlab Prompt: Clear MATLAB Workspaces
      mask DialogControl clear_matlab Callback:
      | command_clear = "clear all";
      |     evalin("base",command_clear)
      mask Display:
      | color('BLUE');
      | 
      | fprintf('Linear System \nand \nModal Analysis');

== system VFlexP/Grid ==
  Dynamic : Subsystem  VariantControl=Dynamic
  Loadflow : Subsystem  VariantControl=Loadflow

== system VFlexP/Modal Analysis ==

== system VFlexP/Grid/Dynamic ==
  Constant2 : Constant  Value=omega_base  VectorParams1D=off
  DCAC converters : Subsystem
  Gain : Gain  Gain=1/(2*pi)
  Gain1 : Gain  Gain=Sb
  Gain2 : Gain  Gain=Sb
  Generators : Subsystem
  Generators_DC : Subsystem
  Goto Tag Visibility : GotoTagVisibility  GotoTag=omega_ref
  Goto Tag Visibility1 : GotoTagVisibility  GotoTag=omega_base
  Grid : Subsystem  Variant=on  VariantControlMode=label  LabelModeActiveChoice=Dynamic
  Grid_DC : Subsystem  Variant=on  VariantControlMode=label  LabelModeActiveChoice=Dynamic
  LPF : Subsystem
  LPF1 : Subsystem
  LPF2 : Subsystem
  LPF3 : Subsystem
  Manual Switch : ManualSwitch
  One : Constant  OutDataTypeStr=Inherit: Inherit via back propagation
  Product1 : Product
  Scope_gen : Scope  NumInputPorts=4
  Secondary Control : Subsystem  Variant=on  VariantControlMode=label  VariantControl=Choice  LabelModeActiveChoice=No SC
      settings: PortSchema="{\"entries\":[{\"content\":{\"sides\":[{\"content\":{\"connectorIds\":[\"Out1\"]},\"type\":\"ConnectorPlacement.EquallySpacedRectSide\",\"uuid\":\"fff1731e-03ae-4532-8327-8c877d5503a1\"},{\"content\":{\"connectorIds\":[\"In1\",\"In2\",\"In3\",\"In4\"],\"side\":\"RIGHT\"},\"type\":\"ConnectorPlacement.EquallySpacedRectSide\",\"uuid\":\"a483b49e-8899-40e0-871c-863b08e1ecd3\"},{\"content\":{\"connectorIds\":[],\"side\":\"TOP\"},\"type\":\"ConnectorPlacement.EquallySpacedRectSide\",\"uuid\":\"d6acdfc2-068d-45c3-a7db-011142f68adc\"},{\"content\":{\"connectorIds\":[],\"side\":\"BOTTOM\"},\"type\":\"ConnectorPlacement.EquallySpacedRectSide\",\"uuid\":\"a007924e-be31-4ab9-87dc-62addce8969f\"}]},\"type\":\"ConnectorPlacement.EquallySpacedConnector\",\"uuid\":\"f40773b4-1769-44e6-aa19-3b4c4e232e75\"}],\"packageUris\":[\"http://schema.mathworks.com/mf0/Connector/R2020b\"],\"version\":\"1.0\"}"
  Selector : Selector  NumberOfDimensions=2  InputPortWidth=3  IndexOptions=Index vector (dialog),Index vector (dialog)  Indices=1,fref.ref_units  OutputSizes=1,1
  Selector1 : Selector  NumberOfDimensions=2  InputPortWidth=3  IndexOptions=Select all,Index vector (dialog)  Indices=[1 3],gen_to_plot  OutputSizes=1,1
  Selector11 : Selector  NumberOfDimensions=2  InputPortWidth=3  IndexOptions=Index vector (dialog),Select all  Indices=4,1  OutputSizes=1,1
  Selector3 : Selector  NumberOfDimensions=2  InputPortWidth=3  IndexOptions=Index vector (dialog),Select all  Indices=2,1  OutputSizes=1,1
  Selector5 : Selector  NumberOfDimensions=2  InputPortWidth=3  IndexOptions=Index vector (dialog),Select all  Indices=3,1  OutputSizes=1,1
  Selector7 : Selector  NumberOfDimensions=2  InputPortWidth=3  IndexOptions=Index vector (dialog),Select all  Indices=1,1  OutputSizes=1,1
  Selector8 : Selector  InputPortWidth=length(fref.ref_units)  IndexOptions=Index vector (dialog)  Indices=fref.Fb_units  OutputSizes=1
  Step : Step  Time=20  SampleTime=0  VectorParams1D=off  ZeroCross=off
  Step1 : Step  Time=10  Before=ones(1, length(buses_lf))  After=[ones(1, length(buses_lf)-1) 1]  SampleTime=0  VectorParams1D=off  ZeroCross=off
  Sum : Sum  Inputs=+++++
  Sum2 : Sum  Inputs=|++
  Tertiary Control : Subsystem  Variant=on  VariantControlMode=label  VariantControl=Choice  LabelModeActiveChoice=No TC
      settings: PortSchema="{\"entries\":[{\"content\":{\"sides\":[{\"content\":{\"connectorIds\":[\"Out1\"]},\"type\":\"ConnectorPlacement.EquallySpacedRectSide\",\"uuid\":\"fff1731e-03ae-4532-8327-8c877d5503a1\"},{\"content\":{\"connectorIds\":[\"In1\",\"In2\",\"In3\"],\"side\":\"RIGHT\"},\"type\":\"ConnectorPlacement.EquallySpacedRectSide\",\"uuid\":\"a483b49e-8899-40e0-871c-863b08e1ecd3\"},{\"content\":{\"connectorIds\":[],\"side\":\"TOP\"},\"type\":\"ConnectorPlacement.EquallySpacedRectSide\",\"uuid\":\"d6acdfc2-068d-45c3-a7db-011142f68adc\"},{\"content\":{\"connectorIds\":[],\"side\":\"BOTTOM\"},\"type\":\"ConnectorPlacement.EquallySpacedRectSide\",\"uuid\":\"a007924e-be31-4ab9-87dc-62addce8969f\"}]},\"type\":\"ConnectorPlacement.EquallySpacedConnector\",\"uuid\":\"f40773b4-1769-44e6-aa19-3b4c4e232e75\"}],\"packageUris\":[\"http://schema.mathworks.com/mf0/Connector/R2020b\"],\"version\":\"1.0\"}"
  To Workspace : ToWorkspace  VariableName=elec  SaveFormat=Timeseries  SampleTime=-1
  iP : Subsystem  Commented=on
  in_current : Subsystem
  in_current_bus : Subsystem
  mod pilot buses1 : Subsystem
  tag scope: omega_base=scoped, omega_ref=scoped
  wires:
  Generators/1(i) -> [i_from_gen]
  [elec] -> Selector/1
  Selector3/1 -> LPF1/1(In1)  "P"
  Selector5/1 -> LPF2/1(In1)  "v"
  Selector11/1 -> LPF3/1(In1)  "Q"
  Secondary Control/1(secondary_refs) -> Generators/2(ref)
  Product1/1 -> Gain/1
  Gain2/1 -> Scope_gen/4  "Q"
  [v_buses] -> Generators/1(v)
  Generators/2(elec) -> To Workspace/1, [elec]
  Selector1/1 -> Selector7/1, Selector11/1, Selector5/1, Selector3/1
  [elec] -> Selector1/1
  [i_from_gen] -> Sum/2
  One/1 -> Manual Switch/2
  Grid_DC/1(v_buses_dc) -> [v_buses_DC]
  [v_buses] -> DCAC converters/1(vac)
  [v_buses_DC] -> DCAC converters/2(vdc)
  Sum/1 -> Grid/1(i_from_gen)
  Step1/1 -> Tertiary Control/1(connect_DGs)
  [elec] -> Tertiary Control/3(elec)
  [v_buses] -> mod pilot buses1/1(v)
  mod pilot buses1/1(vmod) -> Tertiary Control/2(vmod)
  [v_buses] -> Secondary Control/4(v_buses)
  [elec] -> Secondary Control/2(elec)
  Constant2/1 -> [omega_base]
  Selector7/1 -> LPF/1(In1)  "f"
  [omega_base] -> Selector8/1
  Selector8/1 -> Product1/1
  Gain/1 -> Scope_gen/1  "f"
  DCAC converters/2(idc) -> Sum2/1
  Sum2/1 -> Grid_DC/1(i_from_gen_dc)
  Generators_DC/1(i) -> Sum2/2
  [v_buses_DC] -> Generators_DC/1(v)
  DCAC converters/1(iac) -> Sum/4
  Manual Switch/1 -> [omega_ref]
  Selector/1 -> Manual Switch/1
  [v_buses] -> iP/1(v)
  Gain1/1 -> Scope_gen/2  "P"
  Step/1 -> Secondary Control/1(start_SC)
  in_current/1(i) -> Sum/3
  iP/1(i) -> Sum/1
  [v_buses] -> in_current/1(v)
  in_current_bus/1(Out1) -> Sum/5
  Grid/1(v_buses) -> [v_buses]
  LPF/1(Out1) -> Product1/2
  LPF1/1(Out1) -> Gain1/1
  LPF2/1(Out1) -> Scope_gen/3
  LPF3/1(Out1) -> Gain2/1
  Tertiary Control/1(ref) -> Secondary Control/3(tertiary_refs)

== system VFlexP/Grid/Loadflow ==
  Generators : Subsystem
  Goto Tag Visibility : GotoTagVisibility  GotoTag=omega_ref
  Grid : Subsystem  Variant=on  VariantControlMode=label  LabelModeActiveChoice=Dynamic
  Loads : Subsystem
  One : Constant  OutDataTypeStr=Inherit: Inherit via back propagation
  Selector2 : Selector  InputPortWidth=Nbuses  IndexOptions=Index vector (dialog)  Indices=Load_buses  OutputSizes=1
  Selector3 : Selector  InputPortWidth=Nbuses  IndexOptions=Index vector (dialog)  Indices=Load_buses  OutputSizes=1
  to_all_Nodes : Subsystem
  to_all_Nodes1 : Subsystem
  tag scope: omega_ref=scoped
  wires:
  One/1 -> [omega_ref]
  Generators/2(i_q) -> Grid/2(iq_in)
  Generators/1(i_d) -> Grid/1(id_in)
  to_all_Nodes/1(id_out) -> Grid/3(id_out)
  to_all_Nodes1/1(iq_out) -> Grid/4(iq_out)
  Loads/1(id) -> to_all_Nodes/1(In1)
  Loads/2(iq) -> to_all_Nodes1/1(In1)
  Selector2/1 -> Loads/1(vd)
  Selector3/1 -> Loads/2(vq)
  Grid/1(vd) -> Generators/1(vd), Selector2/1
  Grid/2(vq) -> Selector3/1, Generators/2(vq)
